simulink model "RBFNN_1221"  (R2018a)
settings: Solver=FixedStepAuto  StartTime=0.0  StopTime=inf  FixedStep=0.001  RelTol=1e-3  EnableMultiTasking=on
undefined symbols (not defined in the file): HIL, j, qc_get_step_size
libraries: dsparch4 x28, quarc_library x17, simulink x7, vrlib x1
(part 1 of 6)
settings Model: SimulationMode=external  ExtModeTrigDuration=10000  Creator=Administrator  LastModifiedBy=ZJUCZ
settings SolverCC: PositivePriorityOrder=on
settings RTWCC: SystemTargetFile=quarc_win64.tlc  TemplateMakefile=quarc_default_tmf  Description=QUARC Win64 Target
settings STFCustomTargetCC: TargetPreCompLibLocation=C:\PROGRA~3\QUARC\lib\2018a\win64\release  TargetLangStandard=C99 (ISO)  ConcurrentExecutionCompliant=on  SystemTargetFile=quarc_win64.tlc
settings GRTTargetCC: TargetPreCompLibLocation=C:\PROGRA~3\QUARC\lib\2018a\win64\release  ParMdlRefBuildCompliant=off  CompOptLevelCompliant=off  CombineOutputUpdateFcns=off  MatFileLogging=off  CPPClassGenCompliant=off  GRTInterface=on  UseToolchainInfoCompliant=off  ExtMode=on  ExtModeMexFile=quarc_comm

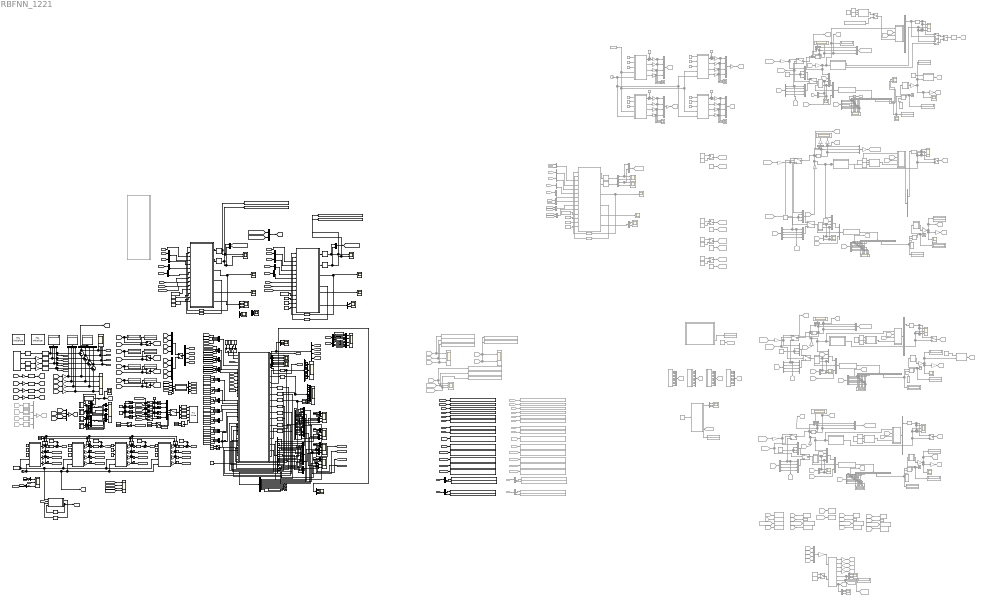
== system RBFNN_1221 ==
  note: 手腕关节的NN控制器
  note: 数据保存区域
  note: 数据传输区
  note: 人工操作区
  note: 轨迹输入区
  note: 向上打是停止运动
  note: 关
      | 节
      | 一
  note: 1关节置零
  note: 关
      | 节
      | 三
  note: 关
      | 节
      | 二
  note: 2关节置零
  note: 3关节置零
  note: 关
      | 节
      | 四
  note: 4关节置零
  note: 左下
  note: 右上
  note: qd
      | e
      | 蓝 FLd QLd
      | 红 FLds1 QLds1
      | 黄 FLda1 QLda1
      | 紫 FLda2 QLda2
      | 绿 QLda3
  note: 主控程序区
  note: 小臂关节的NN控制器
   {,5..7} (4 alike) : Gain  Gain=1/360*2*pi
    {,1..3} (4 alike) : Gain  Commented=on  Gain=1/360*2*pi
     {,1..3} (4 alike) : Gain  Commented=on  Gain=1/360*2*pi
     {4..7} (4 alike) : Gain  Gain=1/360*2*pi
  "  4" : Gain  Commented=on  Gain=-1
  "  5" : Gain  Commented=on
    {6..9} (4 alike) : Gain  Gain=1/360*2*pi
   {1..4} (4 alike) : Gain  Commented=on  Gain=1/360*2*pi
  -25 : Constant  Commented=on  Value=-25
  {1..4} (4 alike) : Gain  Gain=1/360*2*pi
  17.73 : Constant  Commented=on  Value=17.73
  24.22 : Constant  Commented=on  Value=50
  89.3 : Constant  Commented=on  Value=89.3
  Add{,5..7} (4 alike) : Sum  Inputs=++|
  Add{1..4} (4 alike) : Sum  Inputs=+-|
  Analog Filter Design{3..5,7} (4 alike) : dsparch4/Analog Filter Design  Commented=on  method=Butterworth  filttype=Lowpass  N=2  Wlo=30  Whi=80  Rp=2  Rs=40
  Angle from IMU : Subsystem
  Bias : Bias  Bias=-52
  Bias1 : Bias  Bias=+19
  Bias10 : Bias  Bias=-0.5
  Bias11 : Bias  Bias=0.18
  Bias12 : Bias  Bias=0.365
  Bias13 : Bias  Bias=0.21
  Bias14 : Bias  Bias=0.18
  Bias2 : Bias  Bias=-19
  Bias3 : Bias  Bias=-42.6+18+5+2+1-22
  Bias4 : Bias  Bias=-3.5+58
  Bias5 : Bias  Bias=-0.8-1-2
  Bias6 : Bias
  Bias7 : Bias
  Bias8 : Bias  Bias=+0.66
  Bias9 : Bias  Bias=-1.7
  Break : ManualSwitch
  Bus Creator{,1..3} (4 alike) : BusCreator  Commented=on  Inputs=2
  CloseLoop : ManualSwitch  CurrentSetting=0
  Constant{,4..7,11,14,18,31,37,39,44} (12 alike) : Constant  Commented=on  Value=0
  Constant1 : Constant  Commented=on  Value=800
  Constant{2,10,35,41} (4 alike) : Constant  Commented=on  Value=10^3.5
  Constant{12,25,28,60,64,72..73,79..80} (9 alike) : Constant  Value=0
  Constant{3,13,17,36,42} (5 alike) : Constant  Commented=on
  Constant15 : Constant  Value=200-60
  Constant16 : Constant  Commented=on  Value=800
  Constant{9,19,34,40} (4 alike) : Constant  Commented=on  Value=2.5
  Constant20 : Constant  Value=100-50
  Constant21 : Constant  Value=200-50-10
  Constant22 : Constant  Value=100-50
  Constant23 : Constant  Commented=on  Value=-800
  Constant24 : Constant  Value=-0.8
  Constant26 : Constant  Value=-25
  Constant27 : Constant  Value=10
  Constant29 : Constant  Value=5*0
  Constant30 : Constant  Value=0.8
  Constant32 : Constant  Value=100+50
  Constant33 : Constant  Commented=on  Value=800
  Constant38 : Constant  Value=[0;0;0;0]
  Constant43 : Constant  Value=100
  Constant{8,45..46,49,52..53,63,71,78,86} (10 alike) : Constant
  Constant47 : Constant  Value=1e5*5e-3
  Constant48 : Constant  Value=1e5*1e-2
  Constant50 : Constant  Value=1e4
  Constant51 : Constant  Value=1e7
  Constant54 : Constant  Value=100
  Constant55 : Constant  Value=30
  Constant56 : Constant  Value=5e-8
  Constant57 : Constant  Value=6e-8
  Constant58 : Constant  Value=50e-8
  Constant59 : Constant  Value=20e-8
  Constant61 : Constant  Value=240
  Constant62 : Constant  Value=200
  Constant65 : Constant  Value=80
  Constant66 : Constant  Value=80
  Constant67 : Constant  Value=80
  Constant68 : Constant  Value=120
  Constant69 : Constant  Value=100+80+20
  Constant70 : Constant  Value=80-20
  Constant74 : Constant  Commented=on  Value=[5e-7, 8e-4]
  Constant75 : Constant  Commented=on  Value=[ 1, 0.5]
  Constant76 : Constant  Value=3e-3
  Constant77 : Constant  Value=0.5
  Constant81 : Constant  Value=500
  Constant82 : Constant  Commented=on  Value=[1, 1]
  Constant83 : Constant  Commented=on  Value=[500,500]
  Constant84 : Constant  Value=5e-3
  Constant85 : Constant  Value=0.5
  Constant87 : Constant  Value=500
  DIARC_new : MATLAB Function  TreatAsAtomicUnit=on
  Delay : Delay  Commented=on  DelayLength=1
  Delay1 : Delay  DelayLength=1  InitialCondition=[40;60;60;60;25;30;25;20;0;0;0;-10].*2
  Delay10 : Delay  DelayLength=1  InitialCondition=ones(5,1)*0
  Delay11 : Delay  DelayLength=1  InitialCondition=[0,0,0,0,0,0,0,0,0,0,0,0,0,0,0,0,0,0,0,0,0,0,0,0,0,0,0,0,0,0,0,0,0,0,0,0,0]'
  Delay12 : Delay  DelayLength=1  InitialCondition=zeros(5,1)
  Delay13 : Delay  DelayLength=1  InitialCondition=[1e-5,0,0,0,0,0,0,0,0; 0,1e-5,0,0,0,0,0,0,0; 0,0,1e-5,0,0,0,0,0,0; 0,0,0,1e-5,0,0,0,0,0; 0,0,0,0,1e-5,0,0,0,0; 0,0,0,0,0,1e-5,0,0,0; 0,0,0,0,0,0,1e-5,0,0; 0,0,0,0,0,0,0,1e-5,0; 0,0,0,0,0,0,0,0,5e-8]
  Delay{4..5,14..15} (4 alike) : Delay  DelayLength=1  InitialCondition=[0;0;0;0]
  Delay16 : Delay  Commented=on  DelayLength=1  InitialCondition=zeros(5,2)*10-4
  Delay17 : Delay  Commented=on  DelayLength=1  InitialCondition=zeros(5,2)
  Delay18 : Delay  Commented=on  DelayLength=1  InitialCondition=[0,0]
  Delay{3,19,23..24} (4 alike) : Delay  DelayLength=1
  Delay2 : Delay  DelayLength=1  InitialCondition=[0;0;0;0; 0;0;0;0; 2e-10]
  Delay20 : Delay  Commented=on  DelayLength=1  InitialCondition=[0,0]
  Delay21 : Delay  DelayLength=1  InitialCondition=ones(5,1)*1e-4
  Delay22 : Delay  DelayLength=1  InitialCondition=zeros(5,1)
  Delay{6..9} (4 alike) : Delay  DelayLength=1  InitialCondition=[1e-2,0,0; 0,1e-2,0; 0,0,1e-2]
  Demux{,1,3,7} (4 alike) : Demux  Commented=on  Outputs=29
  Demux{2,6,10,18..19,25..28,34,47..48} (12 alike) : Demux
  Demux{11..13,17,49..50} (6 alike) : Demux  Commented=on
  Demux14 : Demux  Commented=on  Outputs=3
  Demux15 : Demux  Commented=on  Outputs=3
  Demux16 : Demux  Commented=on  Outputs=3
  Demux20 : Demux  Outputs=12
  Demux21 : Demux  Outputs=16
  Demux22 : Demux  Outputs=16
  Demux23 : Demux  Outputs=9
  Demux24 : Demux  Outputs=8+4+4
  Demux29 : Demux  Commented=on  Outputs=2
  Demux{30..33,42..45} (8 alike) : Demux  Outputs=[1,1,1,1]
  Demux35 : Demux  Outputs=5
  Demux36 : Demux  Commented=on  Outputs=2
  Demux{37..40} (4 alike) : Demux  Commented=on  Outputs=[1,1,2]
  Demux{4..5,8..9} (4 alike) : Demux  Commented=on  Outputs=27
  Demux41 : Demux  Commented=on  Outputs=2
  Demux46 : Demux  Outputs=2
  Demux51 : Demux  Outputs=5
  Demux52 : Demux  Outputs=5
  Discrete PID Controller1 : simulink/Continuous/PID Controller  Controller=PID  TimeDomain=Continuous-time  SampleTime=-1  IntegratorMethod=Forward Euler  FilterMethod=Backward Euler  Form=Parallel  UseFilter=on  ControllerParametersSource=internal  P=10  I=0  D=0.1  N=2  InitialConditionSource=internal  InitialConditionForIntegrator=0  InitialConditionForFilter=0  ExternalReset=none  IgnoreLimit=on  LimitOutput=off  UpperSaturationLimit=inf  LowerSaturationLimit=-inf  LinearizeAsGain=off  AntiWindupMode=none  Kb=1  TrackingMode=off  Kt=1  PParamMin=[]  PParamMax=[]  IParamMin=[]  IParamMax=[]  DParamMin=[]  DParamMax=[]  NParamMin=[]  NParamMax=[]  KbParamMin=[]  KbParamMax=[]  KtParamMin=[]  KtParamMax=[]  POutMin=[]  POutMax=[]  IOutMin=[]  IOutMax=[]  DOutMin=[]  DOutMax=[]  NOutMin=[]  NOutMax=[]  KbOutMin=[]  KbOutMax=[]  KtOutMin=[]  KtOutMax=[]  IntegratorOutMin=[]  IntegratorOutMax=[]  FilterOutMin=[]  FilterOutMax=[]  SumOutMin=[]  SumOutMax=[]  SumI1OutMin=[]  SumI1OutMax=[]  SumI2OutMin=[]  SumI2OutMax=[]  SumI3OutMin=[]  SumI3OutMax=[]  SumDOutMin=[]  SumDOutMax=[]  SaturationOutMin=[]  SaturationOutMax=[]  IntegratorContinuousStateAttributes=''  IntegratorStateMustResolveToSignalObject=off  IntegratorRTWStateStorageClass=Auto  FilterContinuousStateAttributes=''  FilterStateMustResolveToSignalObject=off  FilterRTWStateStorageClass=Auto  DifferentiatorICPrevScaledInput=0  DifferentiatorOutMin=[]  DifferentiatorOutMax=[]  FilterDiffOutCoefMin=[]  FilterDiffOutCoefMax=[]  SumDenOutMin=[]  SumDenOutMax=[]  SumNumOutMin=[]  SumNumOutMax=[]  ReciprocalOutMin=[]  ReciprocalOutMax=[]  DivideOutMin=[]  DivideOutMax=[]  TunerSelectOption=Transfer Function Based (PID Tuner App)
  Discrete PID Controller2 : simulink/Continuous/PID Controller  Controller=PID  TimeDomain=Continuous-time  SampleTime=-1  IntegratorMethod=Forward Euler  FilterMethod=Backward Euler  Form=Parallel  UseFilter=on  ControllerParametersSource=internal  P=8  I=0  D=0.001  N=1e2  InitialConditionSource=internal  InitialConditionForIntegrator=0  InitialConditionForFilter=0  ExternalReset=none  IgnoreLimit=on  LimitOutput=off  UpperSaturationLimit=inf  LowerSaturationLimit=-inf  LinearizeAsGain=off  AntiWindupMode=none  Kb=1  TrackingMode=off  Kt=1  PParamMin=[]  PParamMax=[]  IParamMin=[]  IParamMax=[]  DParamMin=[]  DParamMax=[]  NParamMin=[]  NParamMax=[]  KbParamMin=[]  KbParamMax=[]  KtParamMin=[]  KtParamMax=[]  POutMin=[]  POutMax=[]  IOutMin=[]  IOutMax=[]  DOutMin=[]  DOutMax=[]  NOutMin=[]  NOutMax=[]  KbOutMin=[]  KbOutMax=[]  KtOutMin=[]  KtOutMax=[]  IntegratorOutMin=[]  IntegratorOutMax=[]  FilterOutMin=[]  FilterOutMax=[]  SumOutMin=[]  SumOutMax=[]  SumI1OutMin=[]  SumI1OutMax=[]  SumI2OutMin=[]  SumI2OutMax=[]  SumI3OutMin=[]  SumI3OutMax=[]  SumDOutMin=[]  SumDOutMax=[]  SaturationOutMin=[]  SaturationOutMax=[]  IntegratorContinuousStateAttributes=''  IntegratorStateMustResolveToSignalObject=off  IntegratorRTWStateStorageClass=Auto  FilterContinuousStateAttributes=''  FilterStateMustResolveToSignalObject=off  FilterRTWStateStorageClass=Auto  DifferentiatorICPrevScaledInput=0  DifferentiatorOutMin=[]  DifferentiatorOutMax=[]  FilterDiffOutCoefMin=[]  FilterDiffOutCoefMax=[]  SumDenOutMin=[]  SumDenOutMax=[]  SumNumOutMin=[]  SumNumOutMax=[]  ReciprocalOutMin=[]  ReciprocalOutMax=[]  DivideOutMin=[]  DivideOutMax=[]  TunerSelectOption=Transfer Function Based (PID Tuner App)
  Discrete PID Controller3 : simulink/Continuous/PID Controller  Controller=PID  TimeDomain=Continuous-time  SampleTime=-1  IntegratorMethod=Forward Euler  FilterMethod=Backward Euler  Form=Parallel  UseFilter=on  ControllerParametersSource=internal  P=15  I=0  D=0.003  N=2  InitialConditionSource=internal  InitialConditionForIntegrator=0  InitialConditionForFilter=0  ExternalReset=none  IgnoreLimit=on  LimitOutput=off  UpperSaturationLimit=inf  LowerSaturationLimit=-inf  LinearizeAsGain=off  AntiWindupMode=none  Kb=1  TrackingMode=off  Kt=1  PParamMin=[]  PParamMax=[]  IParamMin=[]  IParamMax=[]  DParamMin=[]  DParamMax=[]  NParamMin=[]  NParamMax=[]  KbParamMin=[]  KbParamMax=[]  KtParamMin=[]  KtParamMax=[]  POutMin=[]  POutMax=[]  IOutMin=[]  IOutMax=[]  DOutMin=[]  DOutMax=[]  NOutMin=[]  NOutMax=[]  KbOutMin=[]  KbOutMax=[]  KtOutMin=[]  KtOutMax=[]  IntegratorOutMin=[]  IntegratorOutMax=[]  FilterOutMin=[]  FilterOutMax=[]  SumOutMin=[]  SumOutMax=[]  SumI1OutMin=[]  SumI1OutMax=[]  SumI2OutMin=[]  SumI2OutMax=[]  SumI3OutMin=[]  SumI3OutMax=[]  SumDOutMin=[]  SumDOutMax=[]  SaturationOutMin=[]  SaturationOutMax=[]  IntegratorContinuousStateAttributes=''  IntegratorStateMustResolveToSignalObject=off  IntegratorRTWStateStorageClass=Auto  FilterContinuousStateAttributes=''  FilterStateMustResolveToSignalObject=off  FilterRTWStateStorageClass=Auto  DifferentiatorICPrevScaledInput=0  DifferentiatorOutMin=[]  DifferentiatorOutMax=[]  FilterDiffOutCoefMin=[]  FilterDiffOutCoefMax=[]  SumDenOutMin=[]  SumDenOutMax=[]  SumNumOutMin=[]  SumNumOutMax=[]  ReciprocalOutMin=[]  ReciprocalOutMax=[]  DivideOutMin=[]  DivideOutMax=[]  TunerSelectOption=Transfer Function Based (PID Tuner App)
  Discrete PID Controller5 : simulink/Continuous/PID Controller  Controller=PID  TimeDomain=Continuous-time  SampleTime=-1  IntegratorMethod=Forward Euler  FilterMethod=Backward Euler  Form=Parallel  UseFilter=on  ControllerParametersSource=internal  P=5.5  I=0  D=0.003  N=100  InitialConditionSource=internal  InitialConditionForIntegrator=0  InitialConditionForFilter=0  ExternalReset=none  IgnoreLimit=on  LimitOutput=off  UpperSaturationLimit=inf  LowerSaturationLimit=-inf  LinearizeAsGain=off  AntiWindupMode=none  Kb=1  TrackingMode=off  Kt=1  PParamMin=[]  PParamMax=[]  IParamMin=[]  IParamMax=[]  DParamMin=[]  DParamMax=[]  NParamMin=[]  NParamMax=[]  KbParamMin=[]  KbParamMax=[]  KtParamMin=[]  KtParamMax=[]  POutMin=[]  POutMax=[]  IOutMin=[]  IOutMax=[]  DOutMin=[]  DOutMax=[]  NOutMin=[]  NOutMax=[]  KbOutMin=[]  KbOutMax=[]  KtOutMin=[]  KtOutMax=[]  IntegratorOutMin=[]  IntegratorOutMax=[]  FilterOutMin=[]  FilterOutMax=[]  SumOutMin=[]  SumOutMax=[]  SumI1OutMin=[]  SumI1OutMax=[]  SumI2OutMin=[]  SumI2OutMax=[]  SumI3OutMin=[]  SumI3OutMax=[]  SumDOutMin=[]  SumDOutMax=[]  SaturationOutMin=[]  SaturationOutMax=[]  IntegratorContinuousStateAttributes=''  IntegratorStateMustResolveToSignalObject=off  IntegratorRTWStateStorageClass=Auto  FilterContinuousStateAttributes=''  FilterStateMustResolveToSignalObject=off  FilterRTWStateStorageClass=Auto  DifferentiatorICPrevScaledInput=0  DifferentiatorOutMin=[]  DifferentiatorOutMax=[]  FilterDiffOutCoefMin=[]  FilterDiffOutCoefMax=[]  SumDenOutMin=[]  SumDenOutMax=[]  SumNumOutMin=[]  SumNumOutMax=[]  ReciprocalOutMin=[]  ReciprocalOutMax=[]  DivideOutMin=[]  DivideOutMax=[]  TunerSelectOption=Transfer Function Based (PID Tuner App)
  Display{1,8,23,25..27,32..33} (8 alike) : Display
  Display{3,5..6,12..14,16..19,21,24,28..29,31,34} (16 alike) : Display  Commented=on
  Divide{,1..3} (4 alike) : Product  Commented=on  Inputs=*/
  From : From  Commented=on  GotoTag=q1
  From1 : From  Commented=on  GotoTag=QL_1
  From107 : From  Commented=on  GotoTag=q1
  From108 : From  Commented=on  GotoTag=q2
  From109 : From  Commented=on  GotoTag=q3
  From11 : From  Commented=on  GotoTag=dx_3
  From110 : From  Commented=on  GotoTag=q4
  From14 : From  Commented=on  GotoTag=Theta1
  From140 : From  Commented=on  GotoTag=P_i
  From141 : From  Commented=on  GotoTag=P_o
  From142 : From  Commented=on  GotoTag=z2
  From143 : From  Commented=on  GotoTag=z3
  From144 : From  Commented=on  GotoTag=z1
  From149 : From  Commented=on  GotoTag=qd4_dot
  From153 : From  Commented=on  GotoTag=qd4_ddot
  From154 : From  Commented=on  GotoTag=qd4
  From166 : From  Commented=on  GotoTag=z2
  From167 : From  Commented=on  GotoTag=e3
  From168 : From  Commented=on  GotoTag=z3
  From169 : From  Commented=on  GotoTag=P_i
  From17 : From  Commented=on  GotoTag=P1
  From170 : From  Commented=on  GotoTag=P_o
  From171 : From  Commented=on  GotoTag=qd4_dot
  From172 : From  Commented=on  GotoTag=qd3_dddot
  From173 : From  Commented=on  GotoTag=qd3
  From174 : From  Commented=on  GotoTag=e4
  From175 : From  Commented=on  GotoTag=qd4
  From176 : From  Commented=on  GotoTag=qd3_dot
  From177 : From  Commented=on  GotoTag=qd4_dddot
  From19 : From  Commented=on  GotoTag=xv_1
  From199 : From  Commented=on  GotoTag=e3
  From2 : From  Commented=on  GotoTag=q3
  From20 : From  Commented=on  GotoTag=Theta2
  From200 : From  Commented=on  GotoTag=e4
  From201 : From  Commented=on  GotoTag=arc3
  From202 : From  Commented=on  GotoTag=arc4
  From203 : From  Commented=on  GotoTag=joint3_Fld
  From204 : From  Commented=on  GotoTag=joint4_Fld
  From205 : From  Commented=on  GotoTag=joint3_Qld
  From206 : From  Commented=on  GotoTag=joint4_Qld
  From207 : From  Commented=on  GotoTag=q3
  From208 : From  Commented=on  GotoTag=q4
  From209 : From  Commented=on  GotoTag=qd3
  From21 : From  Commented=on  GotoTag=P2
  From210 : From  Commented=on  GotoTag=qd4
  From211 : From  Commented=on  GotoTag=P_i
  From212 : From  Commented=on  GotoTag=P_o
  From213 : From  Commented=on  GotoTag=qd3_dot
  From214 : From  Commented=on  GotoTag=qd4_dot
  From22 : From  Commented=on  GotoTag=tracking_result_2
  From23 : From  Commented=on  GotoTag=xv_2
  From27 : From  Commented=on  GotoTag=dx_1
  From29 : From  Commented=on  GotoTag=QL_3
  From3 : From  Commented=on  GotoTag=Theta1
  From31 : From  Commented=on  GotoTag=Theta3
  From32 : From  Commented=on  GotoTag=Theta3
  From33 : From  Commented=on  GotoTag=P3
  From34 : From  Commented=on  GotoTag=tracking_result_3
  From35 : From  Commented=on  GotoTag=xv_3
  From36 : From  Commented=on  GotoTag=dx_2
  From37 : From  Commented=on  GotoTag=q2
  From38 : From  Commented=on  GotoTag=QL_2
  From40 : From  Commented=on  GotoTag=Theta2
  From50 : From  Commented=on  GotoTag=setzero1
  From51 : From  Commented=on  GotoTag=setzero2
  From52 : From  Commented=on  GotoTag=setzero3
  From57 : From  Commented=on  GotoTag=setvalue1
  From58 : From  Commented=on  GotoTag=setvalue2
  From59 : From  Commented=on  GotoTag=setvalue3
  From60 : From  Commented=on  GotoTag=para1
  From61 : From  Commented=on  GotoTag=para2
  From62 : From  Commented=on  GotoTag=para3
  From63 : From  Commented=on  GotoTag=dx_4
  From64 : From  Commented=on  GotoTag=q4
  From65 : From  Commented=on  GotoTag=QL_4
  From66 : From  Commented=on  GotoTag=Theta4
  From67 : From  Commented=on  GotoTag=setzero4
  From68 : From  Commented=on  GotoTag=setvalue4
  From69 : From  Commented=on  GotoTag=para4
  From74 : From  Commented=on  GotoTag=Theta4
  From75 : From  Commented=on  GotoTag=P4
  From76 : From  Commented=on  GotoTag=tracking_result_4
  From77 : From  Commented=on  GotoTag=xv_4
  From8 : From  Commented=on  GotoTag=tracking_result_1
  From82 : From  Commented=on  GotoTag=errorxyz
  From83 : From  Commented=on  GotoTag=J1_new
  From84 : From  Commented=on  GotoTag=J2_new
  From85 : From  Commented=on  GotoTag=J3_new
  From86 : From  Commented=on  GotoTag=XYZ
  From87 : From  Commented=on  GotoTag=qr4
  From88 : From  Commented=on  GotoTag=qr2
  From89 : From  Commented=on  GotoTag=qr3
  From90 : From  Commented=on  GotoTag=qr1
  From91 : From  Commented=on  GotoTag=J4_new
  Gain{,6..7,16,23,33..36} (9 alike) : Gain  Gain=180/pi
  Gain{1,4,13,20} (4 alike) : Gain  Commented=on
  Gain{3,8..11,15,22,24..28} (12 alike) : Gain  Commented=on  Gain=pi/180
  Gain{12,30..32} (4 alike) : Gain  Gain=-1
  Gain{2,5,14,21} (4 alike) : Gain  Commented=on  Gain=10
  Gain17 : Gain  Commented=on  Gain=-1
  Gain18 : Gain  Commented=on  Gain=-1
  Gain19 : Gain  Commented=on  Gain=-1
  Gain29 : Gain  Commented=on  Gain=180/pi
  Goto : Goto  Commented=on  GotoTag=J1
  Goto10 : Goto  Commented=on  GotoTag=Theta3
  Goto106 : Goto  Commented=on  GotoTag=q_dot
  Goto120 : Goto  Commented=on  GotoTag=RBFNN
  Goto15 : Goto  Commented=on  GotoTag=QL_1
  Goto16 : Goto  Commented=on  GotoTag=dx_1
  Goto17 : Goto  Commented=on  GotoTag=tracking_result_1
  Goto18 : Goto  Commented=on  GotoTag=xv_1
  Goto19 : Goto  Commented=on  GotoTag=tracking_result_3
  Goto20 : Goto  Commented=on  GotoTag=xv_3
  Goto21 : Goto  Commented=on  GotoTag=Theta2
  Goto23 : Goto  Commented=on  GotoTag=QL_3
  Goto24 : Goto  Commented=on  GotoTag=J1_new
  Goto26 : Goto  Commented=on  GotoTag=dx_3
  Goto28 : Goto  Commented=on  GotoTag=tracking_result_2
  Goto29 : Goto  Commented=on  GotoTag=xv_2
  Goto3 : Goto  Commented=on  GotoTag=P1
  Goto30 : Goto  Commented=on  GotoTag=QL_2
  Goto31 : Goto  Commented=on  GotoTag=dx_2
  Goto32 : Goto  Commented=on  GotoTag=P2
  Goto33 : Goto  Commented=on  GotoTag=arc1
  Goto34 : Goto  Commented=on  GotoTag=arc2
  Goto35 : Goto  Commented=on  GotoTag=arc3
  Goto40 : Goto  Commented=on  GotoTag=setzero1
  Goto41 : Goto  Commented=on  GotoTag=setzero2
  Goto42 : Goto  Commented=on  GotoTag=setzero3
  Goto43 : Goto  Commented=on  GotoTag=xd1
  Goto44 : Goto  Commented=on  GotoTag=xd3
  Goto45 : Goto  Commented=on  GotoTag=xd2
  Goto47 : Goto  Commented=on  GotoTag=setvalue1
  Goto48 : Goto  Commented=on  GotoTag=setvalue2
  Goto49 : Goto  Commented=on  GotoTag=setvalue3
  Goto5 : Goto  Commented=on  GotoTag=error
  Goto50 : Goto  Commented=on  GotoTag=para1
  Goto51 : Goto  Commented=on  GotoTag=para2
  Goto52 : Goto  Commented=on  GotoTag=para3
  Goto53 : Goto  Commented=on  GotoTag=Theta4
  Goto54 : Goto  Commented=on  GotoTag=tracking_result_4
  Goto55 : Goto  Commented=on  GotoTag=xv_4
  Goto56 : Goto  Commented=on  GotoTag=QL_4
  Goto57 : Goto  Commented=on  GotoTag=dx_4
  Goto58 : Goto  Commented=on  GotoTag=P4
  Goto59 : Goto  Commented=on  GotoTag=arc4
  Goto60 : Goto  Commented=on  GotoTag=xd4
  Goto62 : Goto  Commented=on  GotoTag=setzero4
  Goto63 : Goto  Commented=on  GotoTag=setvalue4
  Goto67 : Goto  Commented=on  GotoTag=para4
  Goto68 : Goto  Commented=on  GotoTag=J2
  Goto69 : Goto  Commented=on  GotoTag=J3
  Goto7 : Goto  Commented=on  GotoTag=Theta1
  Goto70 : Goto  Commented=on  GotoTag=J4
  Goto71 : Goto  Commented=on  GotoTag=error
  Goto72 : Goto  Commented=on  GotoTag=error
  Goto73 : Goto  Commented=on  GotoTag=XYZ
  Goto74 : Goto  Commented=on  GotoTag=qr1
  Goto75 : Goto  Commented=on  GotoTag=qr2
  Goto76 : Goto  Commented=on  GotoTag=qr3
  Goto77 : Goto  Commented=on  GotoTag=qr4
  Goto78 : Goto  Commented=on  GotoTag=errorxyz
  Goto79 : Goto  Commented=on  GotoTag=e2
  Goto8 : Goto  Commented=on  GotoTag=P3
  Goto80 : Goto  Commented=on  GotoTag=e1
  Goto81 : Goto  Commented=on  GotoTag=e3
  Goto82 : Goto  Commented=on  GotoTag=e4
  Goto83 : Goto  Commented=on  GotoTag=J2_new
  Goto87 : Goto  Commented=on  GotoTag=J3_new
  Goto88 : Goto  Commented=on  GotoTag=J4_new
  HIL Initialize : quarc_library/Data Acquisition/Generic/Configuration/HIL Initialize  object_name=HIL-1  board_type=qpid_e  board_number=0  board_options=enc0_dir=0;enc0_filter=1;enc0_a=1;enc0_b=1;enc0_z=0;enc0_reload=0;enc1_dir=0;enc1_filter=1;enc1_a=1;enc1_b=1;enc1_z=0;enc1_reload=0;enc2_dir=0;enc2_filter=1;enc2_a=1;enc2_b=1;enc2_z=0;enc2_reload=0;enc3_dir=0;enc3_filter=1;enc3_a=1;enc3_b=1;enc3_z=0;enc3_reload=0;enc4_dir=0;enc4_filter=1;enc4_a=1;enc4_b=1;enc4_z=0;enc4_reload=0;enc5_dir=0;enc5_filter=1;enc5_a=1;enc5_b=1;enc5_z=0;enc5_reload=0;enc6_dir=0;enc6_filter=1;enc6_a=1;enc6_b=1;enc6_z=0;enc6_reload=0;enc7_dir=0;enc7_filter=1;enc7_a=1;enc7_b=1;enc7_z=0;enc7_reload=0;ext_int_polarity=0;fuse_polarity=0;convert_polarity=0;watchdog_polarity=0;ext_int_watchdog=0;fuse_watchdog=0;trig1_watchdog=0;watchdog_to_trig1=0;watchdog_to_trig2=0;counter_to_trig0=0;trigger_adcs=0;latch_on_adc=0;pwm_immediate=0  exclusive=off  active=on  hardware_clocks=[0:16]  clock_modes=[]  initial_clock_frequencies=[]  set_clock_params_at_start=off  set_clock_params_at_switch_in=off  set_clock_frequencies_at_start=off  set_clock_frequencies_at_switch_in=off  analog_input_channels=[0:7]  analog_input_configurations=[]  analog_input_maximums=10  analog_input_minimums=-10  set_analog_input_params_at_start=off  set_analog_input_params_at_switch_in=off  analog_output_channels=[0:7]  analog_output_maximums=10  analog_output_minimums=-10  initial_analog_outputs=[0]  final_analog_outputs=[0]  watchdog_analog_outputs=0  set_analog_output_params_at_start=off  set_analog_output_params_at_switch_in=off  set_analog_outputs_at_start=on  set_analog_outputs_at_switch_in=off  set_analog_outputs_at_terminate=on  set_analog_outputs_at_switch_out=off  set_analog_outputs_on_watchdog=off  digital_input_channels=[]  digital_output_channels=[]  digital_output_configuration=[]  initial_digital_outputs=[1]  final_digital_outputs=[1]  watchdog_digital_outputs=[2]  set_digital_output_params_at_start=off  set_digital_output_params_at_switch_in=off  set_digital_outputs_at_start=on  set_digital_outputs_at_switch_in=off  set_digital_outputs_at_terminate=on  set_digital_outputs_at_switch_out=off  set_digital_outputs_on_watchdog=off  encoder_channels=[0:7]  quadrature=[4]  encoder_filter_frequency=40e6/1  initial_encoder_counts=[0]  set_encoder_params_at_start=on  set_encoder_params_at_switch_in=off  set_encoder_counts_at_start=on  set_encoder_counts_at_switch_in=off  pwm_channels=[0:7]  pwm_modes=0  pwm_frequency=40e6/4096  pwm_configuration=[0]  pwm_alignment=[0]  pwm_polarity=[1]  pwm_leading_deadband=[0]  pwm_trailing_deadband=[0]  initial_pwm_outputs=[0]  final_pwm_outputs=[0]  watchdog_pwm_outputs=[0]  set_pwm_params_at_start=on  set_pwm_params_at_switch_in=off  set_pwm_outputs_at_start=on  set_pwm_outputs_at_switch_in=off  set_pwm_outputs_at_terminate=on  set_pwm_outputs_at_switch_out=off  set_pwm_outputs_on_watchdog=off  other_output_channels=[]  initial_other_outputs=[]  final_other_outputs=[]  watchdog_other_outputs=[]  set_other_outputs_at_start=off  set_other_outputs_at_switch_in=off  set_other_outputs_at_terminate=off  set_other_outputs_at_switch_out=off  set_other_outputs_on_watchdog=off
  HIL Initialize2 : quarc_library/Data Acquisition/Generic/Configuration/HIL Initialize  object_name=HIL-2  board_type=q8_usb  board_number=0  board_options=update_rate=fast;ext_int_polarity=0;convert_polarity=1;watchdog_polarity=0;ext_int_watchdog=0;use_convert=0;pwm_immediate=0;decimation=1  exclusive=off  active=on  hardware_clocks=[0:2]  clock_modes=[]  initial_clock_frequencies=[]  set_clock_params_at_start=off  set_clock_params_at_switch_in=off  set_clock_frequencies_at_start=off  set_clock_frequencies_at_switch_in=off  analog_input_channels=[0:7]  analog_input_configurations=[]  analog_input_maximums=10  analog_input_minimums=-10  set_analog_input_params_at_start=on  set_analog_input_params_at_switch_in=off  analog_output_channels=[0:7]  analog_output_maximums=10  analog_output_minimums=-10  initial_analog_outputs=[0]  final_analog_outputs=[0]  watchdog_analog_outputs=0  set_analog_output_params_at_start=on  set_analog_output_params_at_switch_in=off  set_analog_outputs_at_start=on  set_analog_outputs_at_switch_in=off  set_analog_outputs_at_terminate=on  set_analog_outputs_at_switch_out=off  set_analog_outputs_on_watchdog=off  digital_input_channels=[]  digital_output_channels=[]  digital_output_configuration=[]  initial_digital_outputs=[1]  final_digital_outputs=[1]  watchdog_digital_outputs=[1]  set_digital_output_params_at_start=off  set_digital_output_params_at_switch_in=off  set_digital_outputs_at_start=on  set_digital_outputs_at_switch_in=off  set_digital_outputs_at_terminate=on  set_digital_outputs_at_switch_out=off  set_digital_outputs_on_watchdog=off  encoder_channels=[0:7]  quadrature=[4]  encoder_filter_frequency=[]  initial_encoder_counts=[0]  set_encoder_params_at_start=on  set_encoder_params_at_switch_in=off  set_encoder_counts_at_start=on  set_encoder_counts_at_switch_in=off  pwm_channels=[0:7]  pwm_modes=0  pwm_frequency=99.532799999999995e6/4095  pwm_configuration=[0]  pwm_alignment=[0]  pwm_polarity=[1]  pwm_leading_deadband=[0]  pwm_trailing_deadband=[0]  initial_pwm_outputs=[0]  final_pwm_outputs=[0]  watchdog_pwm_outputs=[0]  set_pwm_params_at_start=on  set_pwm_params_at_switch_in=off  set_pwm_outputs_at_start=on  set_pwm_outputs_at_switch_in=off  set_pwm_outputs_at_terminate=on  set_pwm_outputs_at_switch_out=off  set_pwm_outputs_on_watchdog=off  other_output_channels=[]  initial_other_outputs=[]  final_other_outputs=[]  watchdog_other_outputs=[]  set_other_outputs_at_start=off  set_other_outputs_at_switch_in=off  set_other_outputs_at_terminate=off  set_other_outputs_at_switch_out=off  set_other_outputs_on_watchdog=off
  HIL Read Analog : quarc_library/Data Acquisition/Generic/Immediate I//O/HIL Read Analog  object_name=HIL-1  channels=[0]  sample_time=qc_get_step_size  active=on  vector_output=off
  HIL Write : quarc_library/Data Acquisition/Generic/Immediate I//O/HIL Write  object_name=HIL-1  analog_channels=[1:5]  pwm_channels=[]  digital_channels=[]  other_channels=[]  sample_time=-1  active=off  vector_input=off
  J1_P2P(the out is degree°) : MATLAB Function  TreatAsAtomicUnit=on
  J2_P2P(the out is degree°) : MATLAB Function  TreatAsAtomicUnit=on
  J3_P2P(the out is degree°) : MATLAB Function  TreatAsAtomicUnit=on
  J4_P2P(the out is degree°) : MATLAB Function  TreatAsAtomicUnit=on
  K_1 : Mux
  K_2 : Mux
  K_3 : Mux
  Look_J{1..4} (4 alike) : Scope  NumInputPorts=4
  Look_q qdot : Scope  NumInputPorts=4
  Look_q1dot : Scope  NumInputPorts=3
  MATLAB Function : MATLAB Function  Commented=on  TreatAsAtomicUnit=on
  MATLAB Function1 : MATLAB Function  Commented=on  TreatAsAtomicUnit=on
  MATLAB Function10 : MATLAB Function  Commented=on  TreatAsAtomicUnit=on
  MATLAB Function7 : MATLAB Function  Commented=on  TreatAsAtomicUnit=on
  MATLAB Function8 : MATLAB Function  Commented=on  TreatAsAtomicUnit=on
  MATLAB Function9 : MATLAB Function  Commented=on  TreatAsAtomicUnit=on
  MPa2Pa : Gain  Gain=1e6
  MPa2Pa1 : Gain  Gain=1e6
  MPa2Pa2 : Gain  Gain=1e6
  Manual Switch{,1..2,6..7,10,15..16,18} (9 alike) : ManualSwitch  Commented=on
  Manual Switch{5,9,11..13,20} (6 alike) : ManualSwitch  CurrentSetting=0
  Manual Switch14 : ManualSwitch  Commented=on  CurrentSetting=0
  Manual Switch{4,8,17,21..25} (8 alike) : ManualSwitch
  Manual Switch19 : ManualSwitch  Commented=on  CurrentSetting=0
  Manual Switch3 : ManualSwitch  Commented=on  CurrentSetting=0
  Multiply : Product
  Multiply1 : Product
  Mux{,2,7..10,13,18,24..25,34..35,38,59,84} (15 alike) : Mux  Commented=on
  Mux{1,4,11..12,19..21,31} (8 alike) : Mux  Commented=on  Inputs=3
  Mux{6,14,22,32} (4 alike) : Mux  Commented=on  Inputs=7
  Mux{5,15,23,33,86,88..90} (8 alike) : Mux  Commented=on  Inputs=2
  Mux{16..17,26..28,37,39..58,61} (27 alike) : Mux
  Mux{3,29..30,36} (4 alike) : Mux  Commented=on  Inputs=11
  Mux{60,62..72,77..83,85,87} (21 alike) : Mux  Inputs=2
  Mux{73..76} (4 alike) : Mux  Inputs=3
  Nan Switch : Subsystem
  Obs Para Generator1 : MATLAB Function  Commented=on  TreatAsAtomicUnit=on
  Obs Para Generator2 : MATLAB Function  Commented=on  TreatAsAtomicUnit=on
  Obs Para Generator3 : MATLAB Function  Commented=on  TreatAsAtomicUnit=on
  Obs Para Generator4 : MATLAB Function  Commented=on  TreatAsAtomicUnit=on
  P1 : Subsystem
  P2 : Subsystem
  P3 : Subsystem
  P4 : Subsystem
  PID/ARC1 : ManualSwitch  CurrentSetting=0
  PID/ARC2 : ManualSwitch
  PID/ARC3 : ManualSwitch  CurrentSetting=0
  PID/ARC4 : ManualSwitch  CurrentSetting=0
  P_scope1 : Scope  NumInputPorts=4
  P_scope2 : Scope
  Product{,1..15} (16 alike) : Product
  RBFNN_muti : MATLAB Function  Commented=on  TreatAsAtomicUnit=on
  RBFNN_smallarm : MATLAB Function  TreatAsAtomicUnit=on
  RBFNN_wrist : MATLAB Function  TreatAsAtomicUnit=on
  RBFNN_wrist1 : MATLAB Function  Commented=on  TreatAsAtomicUnit=on
  S-Function1 : S-Function  Commented=on  FunctionName=ARC_BACKSTEPPING3  SFunctionDeploymentMode=off  EnableBusSupport=off
  S-Function2 : S-Function  Commented=on  FunctionName=ARC_BACKSTEPPING  SFunctionDeploymentMode=off  EnableBusSupport=off
  S-Function3 : S-Function  Commented=on  FunctionName=ARC_BACKSTEPPING2  SFunctionDeploymentMode=off  EnableBusSupport=off
  S-Function4 : S-Function  Commented=on  FunctionName=ARC_BACKSTEPPING4  SFunctionDeploymentMode=off  EnableBusSupport=off
  Scope{,3..4,12,14,25..27} (8 alike) : Scope  Commented=on  NumInputPorts=2
  Scope{1,13,17,22} (4 alike) : Scope  NumInputPorts=4
  Scope{2,10..11,16,18} (5 alike) : Scope  Commented=on  NumInputPorts=3
  Scope{8..9,15,20,23..24} (6 alike) : Scope  Commented=on
  Scope{7,19,21,28..29} (5 alike) : Scope
  Scope30 : Scope  NumInputPorts=2
  Scope31 : Scope  NumInputPorts=2
  Scope32 : Scope  NumInputPorts=5
  Scope33 : Scope  NumInputPorts=5
  Scope5 : Scope  NumInputPorts=2
  Scope6 : Scope  NumInputPorts=5
  Subsystem : Subsystem  Commented=on
  Subsystem1 : Subsystem  Commented=on
  Subsystem2 : Subsystem  Commented=on
  Subsystem3 : Subsystem  Commented=on
  Subsystem4 : Subsystem  Commented=on
  Subsystem5 : Subsystem  Commented=on
  Subsystem6 : Subsystem  Commented=on
  Subsystem7 : Subsystem  Commented=on
  Subsystem8 : Subsystem  Commented=on
  Subsystem9 : Subsystem  Commented=on
  Sum{1,3,5..6} (4 alike) : Sum  Commented=on  Inputs=+-|
  Switch{,1..4,10,12..13} (8 alike) : Switch  Commented=on  Criteria=u2 ~= 0
  Switch{6..9,11} (5 alike) : Switch
  Switch5 : ManualSwitch  CurrentSetting=0
  To File : ToFile  Commented=on  Filename=tracking_result_1  MatrixName=tracking_result
  To File1 : ToFile  Commented=on  Filename=p_1  MatrixName=p
  To File10 : ToFile  Commented=on  Filename=tracking_result_3  MatrixName=tracking_result
  To File11 : ToFile  Commented=on  Filename=theta_3  MatrixName=theta
  To File12 : ToFile  Commented=on  Filename=xv_3  MatrixName=xv
  To File13 : ToFile  Commented=on  Filename=p_3  MatrixName=p
  To File14 : ToFile  Commented=on  Filename=C:\Users\ZJUCZ\Desktop\RBFNN_EXPERMENT\joint4_e3  MatrixName=joint4_e3
  To File15 : ToFile  Commented=on  Filename=tracking_result_4  MatrixName=tracking_result
  To File16 : ToFile  Commented=on  Filename=theta_4  MatrixName=theta
  To File17 : ToFile  Commented=on  Filename=xv_4  MatrixName=xv
  To File18 : ToFile  Commented=on  Filename=p_4  MatrixName=p
  To File19 : ToFile  Commented=on  Filename=C:\Users\ZJUCZ\Desktop\RBFNN_EXPERMENT\joint4_qd  MatrixName=joint4_qd
  To File2 : ToFile  Commented=on  Filename=theta_1  MatrixName=theta
  To File20 : ToFile  Commented=on  Filename=xyz
  To File21 : ToFile  Commented=on  Filename=errorxyz
  To File22 : ToFile  Commented=on  Filename=C:\Users\ZJUCZ\Desktop\RBFNN_EXPERMENT\joint4_pi  MatrixName=joint4_pi
  To File23 : ToFile  Commented=on  Filename=C:\Users\ZJUCZ\Desktop\RBFNN_EXPERMENT\joint4_po  MatrixName=joint4_po
  To File24 : ToFile  Commented=on  Filename=C:\Users\ZJUCZ\Desktop\RBFNN_EXPERMENT\joint4_qd_dot  MatrixName=joint4_qd_dot
  To File25 : ToFile  Commented=on  Filename=C:\Users\ZJUCZ\Desktop\RBFNN_EXPERMENT\joint4_qd_ddot  MatrixName=joint4_qd_ddot
  To File26 : ToFile  Filename=C:\Users\ZJUCZ\Desktop\RBFNN_EXPERMENT\data\joint_3_nndrc_error.mat  MatrixName=joint_3_nndrc_error
  To File27 : ToFile  Filename=C:\Users\ZJUCZ\Desktop\RBFNN_EXPERMENT\data\joint_4_nndrc_error.mat  MatrixName=joint_4_nndrc_error
  To File28 : ToFile  Filename=C:\Users\ZJUCZ\Desktop\RBFNN_EXPERMENT\data\joint_3_nndrc_qd.mat  MatrixName=joint_3_nndrc_qd
  To File29 : ToFile  Filename=C:\Users\ZJUCZ\Desktop\RBFNN_EXPERMENT\data\joint_4_nndrc_qd.mat  MatrixName=joint_4_nndrc_qd
  To File3 : ToFile  Commented=on  Filename=xv_1  MatrixName=xv
  To File30 : ToFile  Filename=C:\Users\ZJUCZ\Desktop\RBFNN_EXPERMENT\data\joint_4_nndrc_P_i.mat  MatrixName=joint_4_nndrc_P_i
  To File31 : ToFile  Filename=C:\Users\ZJUCZ\Desktop\RBFNN_EXPERMENT\data\joint_3_nndrc_P_i.mat  MatrixName=joint_3_nndrc_P_i
  To File32 : ToFile  Filename=C:\Users\ZJUCZ\Desktop\RBFNN_EXPERMENT\data\joint_4_nndrc_P_o.mat  MatrixName=joint_4_nndrc_P_o
  To File33 : ToFile  Filename=C:\Users\ZJUCZ\Desktop\RBFNN_EXPERMENT\data\joint_3_nndrc_P_o.mat  MatrixName=joint_3_nndrc_P_o
  To File34 : ToFile  Filename=C:\Users\ZJUCZ\Desktop\RBFNN_EXPERMENT\data\joint_3_nndrc_U.mat  MatrixName=joint_3_nndrc_U
  To File35 : ToFile  Filename=C:\Users\ZJUCZ\Desktop\RBFNN_EXPERMENT\data\joint_4_nndrc_U.mat  MatrixName=joint_4_nndrc_U
  To File36 : ToFile  Filename=C:\Users\ZJUCZ\Desktop\RBFNN_EXPERMENT\data\joint_3_nndrc_Fld.mat  MatrixName=joint_3_nndrc_Fld
  To File37 : ToFile  Filename=C:\Users\ZJUCZ\Desktop\RBFNN_EXPERMENT\data\joint_3_nndrc_Qld.mat  MatrixName=joint_3_nndrc_Qld
  To File38 : ToFile  Filename=C:\Users\ZJUCZ\Desktop\RBFNN_EXPERMENT\data\joint_4_nndrc_Fld.mat  MatrixName=joint_4_nndrc_Fld
  To File39 : ToFile  Filename=C:\Users\ZJUCZ\Desktop\RBFNN_EXPERMENT\data\joint_4_nndrc_Qld.mat  MatrixName=joint_4_nndrc_Qld
  To File4 : ToFile  Commented=on  Filename=tracking_result_2  MatrixName=tracking_result
  To File40 : ToFile  Filename=C:\Users\ZJUCZ\Desktop\RBFNN_EXPERMENT\data\joint_3_nndrc_q.mat  MatrixName=joint_3_nndrc_q
  To File41 : ToFile  Filename=C:\Users\ZJUCZ\Desktop\RBFNN_EXPERMENT\data\joint_4_nndrc_q.mat  MatrixName=joint_4_nndrc_q
  To File42 : ToFile  Filename=C:\Users\ZJUCZ\Desktop\RBFNN_EXPERMENT\data\joint_3_nndrc_qddot.mat  MatrixName=joint_3_nndrc_qddot
  To File43 : ToFile  Filename=C:\Users\ZJUCZ\Desktop\RBFNN_EXPERMENT\data\joint_4_nndrc_qddot.mat  MatrixName=joint_4_nndrc_qddot
  To File44 : ToFile  Commented=on  Filename=C:\Users\ZJUCZ\Desktop\RBFNN_EXPERMENT\data\joint_3_drc_error.mat  MatrixName=joint_3_drc_error
  To File45 : ToFile  Commented=on  Filename=C:\Users\ZJUCZ\Desktop\RBFNN_EXPERMENT\data\joint_4_drc_error.mat  MatrixName=joint_4_drc_error
  To File46 : ToFile  Commented=on  Filename=C:\Users\ZJUCZ\Desktop\RBFNN_EXPERMENT\data\joint_3_drc_qd.mat  MatrixName=joint_3_drc_qd
  To File47 : ToFile  Commented=on  Filename=C:\Users\ZJUCZ\Desktop\RBFNN_EXPERMENT\data\joint_4_drc_qd.mat  MatrixName=joint_4_drc_qd
  To File48 : ToFile  Commented=on  Filename=C:\Users\ZJUCZ\Desktop\RBFNN_EXPERMENT\data\joint_4_drc_P_i.mat  MatrixName=joint_4_drc_P_i
  To File49 : ToFile  Commented=on  Filename=C:\Users\ZJUCZ\Desktop\RBFNN_EXPERMENT\data\joint_3_drc_P_i.mat  MatrixName=joint_3_drc_P_i
  To File5 : ToFile  Commented=on  Filename=theta_2  MatrixName=theta
  To File50 : ToFile  Commented=on  Filename=C:\Users\ZJUCZ\Desktop\RBFNN_EXPERMENT\data\joint_4_drc_P_o.mat  MatrixName=joint_4_drc_P_o
  To File51 : ToFile  Commented=on  Filename=C:\Users\ZJUCZ\Desktop\RBFNN_EXPERMENT\data\joint_3_drc_P_o.mat  MatrixName=joint_3_drc_P_o
  To File52 : ToFile  Commented=on  Filename=C:\Users\ZJUCZ\Desktop\RBFNN_EXPERMENT\data\joint_3_drc_U.mat  MatrixName=joint_3_drc_U
  To File53 : ToFile  Commented=on  Filename=C:\Users\ZJUCZ\Desktop\RBFNN_EXPERMENT\data\joint_4_drc_U.mat  MatrixName=joint_4_drc_U
  To File54 : ToFile  Commented=on  Filename=C:\Users\ZJUCZ\Desktop\RBFNN_EXPERMENT\data\joint_3_drc_Fld.mat  MatrixName=joint_3_drc_Fld
  To File55 : ToFile  Commented=on  Filename=C:\Users\ZJUCZ\Desktop\RBFNN_EXPERMENT\data\joint_3_drc_Qld.mat  MatrixName=joint_3_drc_Qld
  To File56 : ToFile  Commented=on  Filename=C:\Users\ZJUCZ\Desktop\RBFNN_EXPERMENT\data\joint_4_drc_Fld.mat  MatrixName=joint_4_drc_Fld
  To File57 : ToFile  Commented=on  Filename=C:\Users\ZJUCZ\Desktop\RBFNN_EXPERMENT\data\joint_4_drc_Qld.mat  MatrixName=joint_4_drc_Qld
  To File58 : ToFile  Commented=on  Filename=C:\Users\ZJUCZ\Desktop\RBFNN_EXPERMENT\data\joint_3_drc_q.mat  MatrixName=joint_3_drc_q
  To File59 : ToFile  Commented=on  Filename=C:\Users\ZJUCZ\Desktop\RBFNN_EXPERMENT\data\joint_4_drc_q.mat  MatrixName=joint_4_drc_q
  To File6 : ToFile  Commented=on  Filename=xv_2  MatrixName=xv
  To File60 : ToFile  Commented=on  Filename=C:\Users\ZJUCZ\Desktop\RBFNN_EXPERMENT\data\joint_3_drc_qddot.mat  MatrixName=joint_3_drc_qddot
  To File61 : ToFile  Commented=on  Filename=C:\Users\ZJUCZ\Desktop\RBFNN_EXPERMENT\data\joint_4_drc_qddot.mat  MatrixName=joint_4_drc_qddot
  To File62 : ToFile  Filename=C:\Users\ZJUCZ\Desktop\RBFNN_EXPERMENT\data\joint_3_nndrc_Fnn.mat  MatrixName=joint_3_nndrc_Fnn
  To File63 : ToFile  Filename=C:\Users\ZJUCZ\Desktop\RBFNN_EXPERMENT\data\joint_3_nndrc_Qnn.mat  MatrixName=joint_3_nndrc_Qnn
  To File66 : ToFile  Filename=C:\Users\ZJUCZ\Desktop\RBFNN_EXPERMENT\data\joint_4_nndrc_Fnn.mat  MatrixName=joint_4_nndrc_Fnn
  To File67 : ToFile  Filename=C:\Users\ZJUCZ\Desktop\RBFNN_EXPERMENT\data\joint_4_nndrc_Qnn.mat  MatrixName=joint_4_nndrc_Qnn
  To File7 : ToFile  Commented=on  Filename=p_2  MatrixName=p
  To File8 : ToFile  Commented=on  Filename=C:\Users\ZJUCZ\Desktop\RBFNN_EXPERMENT\joint4_e1  MatrixName=joint4_e1
  To File9 : ToFile  Commented=on  Filename=C:\Users\ZJUCZ\Desktop\RBFNN_EXPERMENT\joint4_e2  MatrixName=joint4_e2
  Unit Delay : UnitDelay  Commented=on  SampleTime=-1
  VS Communication (Visual Signal) : Subsystem  Commented=on
  bias{,1..3} (4 alike) : Sum  Commented=on  Inputs=++|
  break : Constant  Value=-1
  break1 : Constant
  close loop : Constant  Value=-1
  constant Velocity (m/s)1 : Constant  Commented=on  Value=0
  controller parameter1 : Subsystem  Commented=on
  controller parameter3 : Subsystem  Commented=on
  controller parameter4 : Subsystem  Commented=on
  controller parameter5 : Subsystem  Commented=on
  degree2rad{,1..3,9} (5 alike) : Gain  Commented=on  Gain=1/360*2*pi
  degree2rad10 : Gain  Gain=-1/360*2*pi
  degree2rad{4..8,11..12} (7 alike) : Gain  Gain=1/360*2*pi
  degree2rad13 : Gain  Gain=-1/360*2*pi
  dx_{1..4} (4 alike) : Scope  Commented=on  NumInputPorts=3
  e1_scope : Scope  NumInputPorts=4
  e2_scope : Scope  NumInputPorts=4
  e3_scope : Scope  NumInputPorts=4
  e=q-qd : Display
  g_d1 : Mux
  g_d2 : Mux
  gripper : ManualSwitch  CurrentSetting=0
  ini_bias : Constant  Commented=on  Value=0
  ini_bias1 : Constant  Commented=on  Value=10
  ini_bias2 : Constant  Commented=on  Value=60
  ini_bias3 : Constant  Commented=on  Value=0
  k_obs4 : Constant  Commented=on  Value=[1*10^2.5;5*10^4.2;2*10^6.3]  VectorParams1D=off
  limit_u : MATLAB Function  Commented=on  TreatAsAtomicUnit=on
  limit_u1 : MATLAB Function  Commented=on  TreatAsAtomicUnit=on
  limit_u2 : MATLAB Function  Commented=on  TreatAsAtomicUnit=on
  limit_u3 : MATLAB Function  Commented=on  TreatAsAtomicUnit=on
  look_e1 : Scope  NumInputPorts=4
  open loop : Constant  Value=0
  pin_pout : Scope  Commented=on  NumInputPorts=2
  pressure detect : Subsystem  Commented=on
  pressure detect1 : Subsystem  Commented=on
  pressure detect2 : Subsystem  Commented=on
  pressure detect3 : Subsystem  Commented=on
  q,qd,qdd,qddd{,1..3} (4 alike) : Mux  Commented=on
  q2qfdot_rad : MATLAB Function  TreatAsAtomicUnit=on
  qd{,1..3} (4 alike) : Scope  Commented=on  NumInputPorts=4
  "qd " : Display
  qd(°){,1..3} (4 alike) : Constant  Commented=on  Value=40
  qd(°){4..7} (4 alike) : Constant  Value=40
  qd_ddot{,1..3} (4 alike) : Constant  Commented=on  Value=20
  qd_ddot{4..7} (4 alike) : Constant  Value=30
  qd_dot{,1..3} (4 alike) : Constant  Commented=on  Value=20
  qd_dot{4..7} (4 alike) : Constant  Value=30
  qd_scope : Scope  NumInputPorts=4
  qr : Display
  rad2degree : Gain  Gain=2*pi/360
  run : Constant  Value=0
  run1 : Constant  Value=0
  t : Clock  Commented=on
  t1 : Clock
  theta{,1..3} (4 alike) : Scope  Commented=on  NumInputPorts=7
  "theta_s1_scope " : Scope  NumInputPorts=3
  "theta_s2_scope " : Scope  NumInputPorts=3
  ts : Constant  Commented=on  Value=0.001
  ts1 : Constant  Value=0.001
  u{,1..3} (4 alike) : Scope  Commented=on
  velocity caculator : Subsystem  Commented=on
  velocity caculator1 : Subsystem  Commented=on
  velocity caculator2 : Subsystem  Commented=on
  velocity caculator3 : Subsystem  Commented=on
  velocity caculator4 : Subsystem  Commented=on
  velocity caculator5 : Subsystem  Commented=on
  velocity caculator6 : Subsystem  Commented=on
  velocity caculator7 : Subsystem  Commented=on
  w2 : Mux
  w3 : Mux
  x{1..4} (4 alike) : Scope  Commented=on  NumInputPorts=2
  xv : Scope  Commented=on
  一键ARC : ManualSwitch
  置零{,1..3} (4 alike) : Constant  Commented=on
  wires:
  Bus Creator/1 -> x1/1
  Mux1/1 -> S-Function2/1
  Mux/1 -> Mux1/1
  velocity caculator/1(dxr) -> Manual Switch14/1, Sum3/2, dx_1/2
  pressure detect/1(pin) -> pin_pout/1, Mux5/1, Mux/3
  S-Function2/1 -> Demux/1
  Divide/1 -> Display3/1, limit_u/1(u), u/1
  Mux2/1 -> Switch2/3
  Mux7/1 -> Switch2/1
  Switch2/1 -> Mux1/2
  Constant1/1 -> Divide/2
  置零/1 -> Manual Switch3/1
  Constant6/1 -> Manual Switch3/2
  Constant7/1 -> Mux7/2, Mux7/4, Mux7/3
  From57/1 -> Gain10/1
  From/1 -> Gain9/1
  Demux/2 -> Mux6/2, theta/2
  Demux/4 -> Mux6/4, theta/4
  Demux/5 -> Mux6/5, theta/5
  Demux/6 -> Mux6/6, theta/6
  Demux/1 -> Mux6/1, theta/1
  Demux/8 -> Unit Delay/1
  Demux/18 -> Display6/1, Divide/1, xv/1
  pressure detect/2(pout) -> Mux5/2, pin_pout/2, Mux/4
  Mux5/1 -> Goto3/1
  Demux/3 -> Mux6/3, theta/3
  Demux/7 -> Mux6/7, theta/7
  Mux6/1 -> Goto7/1
  limit_u/1(y) -> Gain1/1
  From59/1 -> Gain11/1
  Mux8/1 -> Switch3/3
  Constant14/1 -> Mux9/2, Mux9/4, Mux9/3
  Mux9/1 -> Switch3/1
  From2/1 -> Gain8/1
  Bus Creator1/1 -> x2/1
  Mux10/1 -> Mux12/1
  Switch3/1 -> Mux12/2
  Mux12/1 -> S-Function1/1
  Demux1/2 -> Mux14/2, theta1/2
  S-Function1/1 -> Demux1/1
  Demux1/4 -> Mux14/4, theta1/4
  Mux14/1 -> Goto10/1
  Demux1/7 -> Mux14/7, theta1/7
  Demux1/3 -> Mux14/3, theta1/3
  Demux1/8 -> Goto23/1
  Demux1/1 -> Mux14/1, theta1/1
  Demux1/5 -> Mux14/5, theta1/5
  Demux1/6 -> Mux14/6, theta1/6
  Divide1/1 -> Display13/1, limit_u1/1(u), u1/1
  Constant16/1 -> Divide1/2
  Demux1/18 -> Display14/1, Divide1/1
  limit_u1/1(y) -> Gain4/1
  Mux15/1 -> Goto8/1
  pressure detect1/1(pin) -> Mux10/3, Scope/1, Mux15/1
  pressure detect1/2(pout) -> Mux15/2, Scope/2, Mux10/4
  Mux16/1 -> qr/1
  Angle from IMU/1(q1) -> Bias/1
  Angle from IMU/2(q2) -> Gain30/1
  Constant79/1 -> Nan Switch/2(angle signal)
  [control2] -> Mux17/2
  Mux17/1 -> Nan Switch/1(control input)
  [control1] -> Mux17/1
  Nan Switch/1(control) -> Demux2/1
  VS Communication (Visual Signal)/3(Error) -> Display19/1
  Gain10/1 -> Mux7/1, Switch/1
  Gain11/1 -> Switch1/1, Mux9/1
  Angle from IMU/3("q3 ") -> Bias1/1
  Angle from IMU/4(q4) -> Bias2/1
  Bias/1 -> Bias6/1
  Constant25/1 -> Switch5/1, Manual Switch11/1, Manual Switch8/1, Manual Switch4/1
  Constant30/1 -> Manual Switch5/1, Manual Switch12/1, Manual Switch13/1, Manual Switch9/1
  Switch9/1 -> Switch5/2
  Switch6/1 -> Manual Switch4/2
  [Control4] -> Switch9/3
  [Control3] -> Switch8/3
  [Control2] -> Switch7/3
  Manual Switch9/1 -> Switch7/1
  Manual Switch13/1 -> Switch8/1
  Switch7/1 -> Manual Switch8/2
  Manual Switch5/1 -> Switch6/1
  Bias12/1 -> HIL Write/2
  Gain12/1 -> Switch9/1
  Bias13/1 -> HIL Write/4
  [Switch_Val] -> Switch9/2, Switch8/2, Switch7/2, Switch6/2
  [Control1] -> Switch6/3
  Switch8/1 -> Manual Switch11/2
  Bias14/1 -> HIL Write/3
  Constant24/1 -> Manual Switch12/2, Manual Switch5/2, Manual Switch9/2, Manual Switch13/2
  Manual Switch12/1 -> Gain12/1
  close loop/1 -> CloseLoop/2
  CloseLoop/1 -> [Switch_Val]
  open loop/1 -> CloseLoop/1
  Unit Delay/1 -> Goto15/1
  From3/1 -> Subsystem/3(theta)
  Subsystem/1(Output) -> Demux9/1
  Demux9/5 -> Manual Switch7/2, Analog Filter Design3/1
  Sum3/1 -> dx_1/3
  Mux4/1 -> Goto17/1
  Gain2/1 -> Goto18/1
  Mux11/1 -> Goto19/1
  Gain5/1 -> Goto20/1
  From14/1 -> To File2/1
  From17/1 -> To File1/1
  From8/1 -> To File/1
  From19/1 -> To File3/1
  From22/1 -> To File4/1
  From21/1 -> To File7/1
  From20/1 -> To File5/1
  From23/1 -> To File6/1
  Obs Para Generator1/1(k_obs) -> Manual Switch2/1
  k_obs4/1 -> Manual Switch2/2
  Constant10/1 -> Obs Para Generator1/2(gain)
  Manual Switch2/1 -> Subsystem/4(k_obs)
  Constant9/1 -> Obs Para Generator1/1(a)
  Analog Filter Design3/1 -> Manual Switch7/1, Sum3/1, dx_1/1
  Constant17/1 -> Obs Para Generator1/3(th)
  From27/1 -> Mux/2
  Constant18/1 -> MATLAB Function/1(bias)
  MATLAB Function/1(out) -> Goto33/1
  Demux/28 -> Scope12/1
  Demux/29 -> Scope12/2
  From1/1 -> Subsystem/2(u)
  Gain9/1 -> Subsystem2/2(xr), Mux/1, velocity caculator/1(xr), Subsystem/1(xp), Display5/1
  Discrete PID Controller1/1 -> [PIDJ1]
  [PIDJ1] -> PID/ARC1/1, Display1/1
  Switch/1 -> Subsystem2/1(xd), Mux4/1, Bus Creator/1
  Subsystem2/1(qr) -> Goto74/1, Mux4/2, Bus Creator/2
  Subsystem2/2(e) -> x1/2, Goto80/1, Mux4/3
  Switch1/1 -> Mux11/1, Bus Creator1/1, Subsystem3/1(xd)
  Subsystem3/1(qr) -> Mux11/2, Bus Creator1/2, Goto76/1
  Sum1/1 -> dx_3/3
  velocity caculator1/1(dxr) -> dx_3/2, Sum1/2, Manual Switch10/2
  Obs Para Generator2/1(k_obs) -> Subsystem4/4(k_obs)
  Demux4/5 -> Analog Filter Design4/1
  From29/1 -> Subsystem4/2(u)
  Gain8/1 -> Subsystem3/2(xr), Mux10/1, Subsystem4/1(xp), velocity caculator1/1(xr)
  Manual Switch10/1 -> Goto26/1
  Analog Filter Design4/1 -> Manual Switch10/1, Sum1/1, dx_3/1
  From31/1 -> Subsystem4/3(theta)
  Subsystem4/1(Output) -> Demux4/1
  Constant2/1 -> Obs Para Generator2/2(gain)
  Constant19/1 -> Obs Para Generator2/1(a)
  Constant3/1 -> Obs Para Generator2/3(th)
  From11/1 -> Mux10/2
  From34/1 -> To File10/1
  From33/1 -> To File13/1
  From32/1 -> To File11/1
  From35/1 -> To File12/1
  Constant35/1 -> Obs Para Generator3/2(gain)
  Obs Para Generator3/1(k_obs) -> Subsystem5/4(k_obs)
  Subsystem1/2(e) -> Goto79/1, Gain18/1, Mux19/3
  Switch4/1 -> Mux19/1, Bus Creator2/1, Subsystem1/1(xd)
  Gain14/1 -> Goto29/1
  Subsystem1/1(qr) -> Mux19/2, Goto75/1, Bus Creator2/2
  Gain15/1 -> Subsystem1/2(xr), Mux13/1, Subsystem5/1(xp), velocity caculator2/1(xr)
  Divide2/1 -> Display12/1, limit_u2/1(u), u2/1
  velocity caculator2/1(dxr) -> dx_2/2, Sum5/2, Manual Switch15/2
  Demux3/8 -> Goto30/1
  Demux3/3 -> Mux22/3, theta2/3
  Mux19/1 -> Gain19/1
  Bus Creator2/1 -> Gain17/1
  Switch10/1 -> Mux20/2
  limit_u2/1(y) -> Gain13/1
  Demux3/1 -> Mux22/1, theta2/1
  Demux3/2 -> Mux22/2, theta2/2
  pressure detect2/2(pout) -> Mux23/2, Scope14/2, Mux13/4
  Constant34/1 -> Obs Para Generator3/1(a)
  pressure detect2/1(pin) -> Mux13/3, Scope14/1, Mux23/1
  Mux23/1 -> Goto32/1
  Demux3/18 -> Display16/1, Divide2/1
  From58/1 -> Gain3/1
  Gain13/1 -> Goto34/1, Display21/1, Scope20/1, Gain14/1
  Constant33/1 -> Divide2/2
  Demux3/6 -> Mux22/6, theta2/6
  Mux24/1 -> Switch10/3
  S-Function3/1 -> Demux3/1
  Demux3/4 -> Mux22/4, theta2/4
  Constant31/1 -> Mux25/2, Mux25/4, Mux25/3
  Mux22/1 -> Goto21/1
  Gain3/1 -> Switch4/1, Mux25/1
  From37/1 -> Gain15/1
  Mux20/1 -> S-Function3/1
  Constant36/1 -> Obs Para Generator3/3(th)
  Analog Filter Design5/1 -> dx_2/1, Manual Switch15/1, Sum5/1
  Demux3/5 -> Mux22/5, theta2/5
  Demux5/5 -> Analog Filter Design5/1
  Demux3/7 -> Mux22/7, theta2/7
  Mux13/1 -> Mux20/1
  From40/1 -> Subsystem5/3(theta)
  From38/1 -> Subsystem5/2(u)
  Mux25/1 -> Switch10/1
  Subsystem5/1(Output) -> Demux5/1
  Manual Switch15/1 -> Goto31/1
  Sum5/1 -> dx_2/3
  From36/1 -> Mux13/2
  Discrete PID Controller5/1 -> [pid2]
  Subsystem3/2(e) -> Goto81/1, x2/2, Mux11/3
  [arc1] -> PID/ARC1/2, Display23/1
  [pid2] -> PID/ARC2/1, Display8/1
  [arc2] -> Display25/1, PID/ARC2/2
  Gain4/1 -> Display18/1, MATLAB Function1/2(xv), Scope9/1, Gain5/1
  MATLAB Function1/1(out) -> Goto35/1
  Constant37/1 -> MATLAB Function1/1(bias)
  [pid3] -> Display26/1, PID/ARC3/1
  [arc3] -> Display27/1, PID/ARC3/2
  [temp2] -> Mux26/2
  [temp3] -> Mux26/3
  [temp1] -> Mux26/1
  [arc1] -> Mux27/1
  [pid2] -> Mux27/2
  [arc3] -> Mux27/3
  Demux6/1 -> [Control1]
  Demux6/2 -> [Control2]
  Demux6/3 -> [Control3]
  Mux26/1 -> 一键ARC/1
  Mux27/1 -> 一键ARC/2
  Demux6/4 -> [Control4]
  [temp4] -> Mux26/4
  [arc4] -> Mux27/4
  From50/1 -> Switch/2, Switch2/2
  Manual Switch3/1 -> Goto40/1
  Constant5/1 -> Manual Switch18/2
  置零2/1 -> Manual Switch18/1
  Manual Switch18/1 -> Goto41/1
  Manual Switch19/1 -> Goto42/1
  置零3/1 -> Manual Switch19/1
  Constant39/1 -> Manual Switch19/2
  From51/1 -> Switch10/2, Switch4/2
  From52/1 -> Switch3/2, Switch1/2
  Mux28/1 -> "qd "/1
  [qd1] -> Gain/1
  [qd3] -> Gain16/1
  [qd2] -> Gain6/1
  Gain/1 -> qd_scope/1, Add1/2, Mux28/1
  Gain16/1 -> qd_scope/3, Add3/2, Mux28/3
  [qd4] -> Gain23/1
  17.73/1 -> Goto47/1
  -25/1 -> Goto48/1
  89.3/1 -> Goto49/1
  controller parameter3/9(gam6) -> Mux29/9
  controller parameter3/6(gam3) -> Mux29/6
  controller parameter3/11(gam8) -> Mux29/11
  controller parameter3/8(gam5) -> Mux29/8
  Mux29/1 -> Goto50/1
  controller parameter3/10(gam7) -> Mux29/10
  controller parameter3/4(gam1) -> Mux29/4
  controller parameter3/3(k3) -> Mux29/3
  controller parameter3/2(k2) -> Mux29/2
  controller parameter3/7(gam4) -> Mux29/7
  controller parameter3/5(gam2) -> Mux29/5
  controller parameter3/1(k1) -> Mux29/1
  From60/1 -> Mux1/3
  Mux3/1 -> Goto51/1
  controller parameter4/1(k1) -> Mux3/1
  controller parameter4/7(gam4) -> Mux3/7
  controller parameter4/5(gam2) -> Mux3/5
  controller parameter4/3(k3) -> Mux3/3
  controller parameter4/2(k2) -> Mux3/2
  controller parameter4/4(gam1) -> Mux3/4
  controller parameter4/10(gam7) -> Mux3/10
  controller parameter4/6(gam3) -> Mux3/6
  controller parameter4/11(gam8) -> Mux3/11
  controller parameter4/9(gam6) -> Mux3/9
  controller parameter4/8(gam5) -> Mux3/8
  controller parameter5/9(gam6) -> Mux30/9
  controller parameter5/8(gam5) -> Mux30/8
  controller parameter5/7(gam4) -> Mux30/7
  controller parameter5/4(gam1) -> Mux30/4
  controller parameter5/6(gam3) -> Mux30/6
  controller parameter5/11(gam8) -> Mux30/11
  controller parameter5/2(k2) -> Mux30/2
  controller parameter5/10(gam7) -> Mux30/10
  controller parameter5/3(k3) -> Mux30/3
  Mux30/1 -> Goto52/1
  controller parameter5/5(gam2) -> Mux30/5
  controller parameter5/1(k1) -> Mux30/1
  From61/1 -> Mux20/3
  From62/1 -> Mux12/3
  Gain17/1 -> x3/1
  Gain18/1 -> x3/2
  Gain19/1 -> Goto28/1
  Mux21/1 -> Goto54/1
  Demux7/8 -> Goto56/1
  Gain20/1 -> Goto59/1, Display31/1, Scope15/1, Gain21/1
  From64/1 -> Gain22/1
  From69/1 -> Mux31/3
  S-Function4/1 -> Demux7/1
  Analog Filter Design7/1 -> Manual Switch1/1, Sum6/1, dx_4/1
  limit_u3/1(y) -> Gain20/1
  Demux8/5 -> Analog Filter Design7/1
  Mux18/1 -> Mux31/1
  From67/1 -> Switch12/2, Switch13/2
  Switch12/1 -> Mux31/2
  Mux35/1 -> Switch12/1
  Mux34/1 -> Switch12/3
  pressure detect3/1(pin) -> Mux18/3, Scope4/1, Mux33/1
  Demux7/5 -> Mux32/5, theta3/5
  Bus Creator3/1 -> x4/1
  Demux7/1 -> Mux32/1, theta3/1
  velocity caculator3/1(dxr) -> dx_4/2, Sum6/2, Manual Switch1/2
  Demux7/6 -> Mux32/6, theta3/6
  Obs Para Generator4/1(k_obs) -> Subsystem7/4(k_obs)
  Mux31/1 -> S-Function4/1
  From63/1 -> Mux18/2
  Subsystem7/1(Output) -> Demux8/1
  Divide3/1 -> Display28/1, limit_u3/1(u), u3/1
  Sum6/1 -> dx_4/3
  Demux7/7 -> Mux32/7, theta3/7
  Manual Switch1/1 -> Goto57/1
  From66/1 -> Subsystem7/3(theta)
  Demux7/4 -> Mux32/4, theta3/4
  Constant11/1 -> Mux35/2, Mux35/4, Mux35/3
  Constant23/1 -> Divide3/2
  From68/1 -> Gain26/1
  Demux7/3 -> Mux32/3, theta3/3
  Demux7/2 -> Mux32/2, theta3/2
  pressure detect3/2(pout) -> Mux33/2, Scope4/2, Mux18/4
  From65/1 -> Subsystem7/2(u)
  Mux33/1 -> Goto58/1
  Gain26/1 -> Switch13/1, Mux35/1
  Constant40/1 -> Obs Para Generator4/1(a)
  Mux32/1 -> Goto53/1
  Subsystem6/1(qr) -> Goto77/1, Bus Creator3/2, Mux21/2
  Demux7/18 -> Display29/1, Divide3/1
  Gain21/1 -> Goto55/1
  Switch13/1 -> Mux21/1, Bus Creator3/1, Subsystem6/1(xd)
  Constant42/1 -> Obs Para Generator4/3(th)
  Constant41/1 -> Obs Para Generator4/2(gain)
  Gain22/1 -> Subsystem6/2(xr), Mux18/1, Subsystem7/1(xp), velocity caculator3/1(xr)
  24.22/1 -> Goto63/1
  Manual Switch6/1 -> Goto62/1
  置零1/1 -> Manual Switch6/1
  [arc4] -> Display33/1, PID/ARC4/2
  [pid4] -> Display32/1, PID/ARC4/1
  Constant44/1 -> Manual Switch6/2
  Demux2/1 -> [temp1]
  Demux2/2 -> [temp2]
  Demux2/3 -> [temp3]
  Demux2/4 -> [temp4]
  PID/ARC1/1 -> [control1]
  PID/ARC4/1 -> [control4]
  PID/ARC3/1 -> [control3]
  PID/ARC2/1 -> [control2]
  [control3] -> Mux17/3
  [control4] -> Mux17/4
  From74/1 -> To File16/1
  From76/1 -> To File15/1
  From75/1 -> To File18/1
  From77/1 -> To File17/1
  controller parameter1/1(k1) -> Mux36/1
  Mux36/1 -> Goto67/1
  controller parameter1/5(gam2) -> Mux36/5
  controller parameter1/10(gam7) -> Mux36/10
  controller parameter1/6(gam3) -> Mux36/6
  controller parameter1/7(gam4) -> Mux36/7
  controller parameter1/11(gam8) -> Mux36/11
  controller parameter1/4(gam1) -> Mux36/4
  controller parameter1/8(gam5) -> Mux36/8
  controller parameter1/9(gam6) -> Mux36/9
  controller parameter1/3(k3) -> Mux36/3
  controller parameter1/2(k2) -> Mux36/2
  Gain23/1 -> qd_scope/4, Add4/2, Mux28/4
  constant Velocity (m/s)1/1 -> Subsystem8/1(In1)
  Subsystem8/1(xyz) -> Demux14/1
  Demux14/1 -> Scope10/1
  Demux14/2 -> Scope10/2
  Demux14/3 -> Scope10/3
  Subsystem8/6(J5) -> Display24/1, Goto5/1
  Constant4/1 -> Goto71/1
  From86/1 -> To File20/1
  From82/1 -> To File21/1
  Demux17/1 -> Goto60/1, Mux34/1, Switch13/3
  velocity caculator/2(dxb) -> Manual Switch14/2
  Manual Switch16/1 -> Delay/1
  Manual Switch7/1 -> Manual Switch16/1
  Manual Switch14/1 -> Manual Switch16/2
  Delay/1 -> Goto16/1
  Demux11/1 -> Goto43/1, Switch/3, Mux2/1
  Gain1/1 -> Scope8/1, Gain2/1, MATLAB Function/2(xv), Display17/1
  Demux12/1 -> Goto44/1, Mux8/1, Switch1/3
  Demux13/1 -> Goto45/1, Mux24/1, Switch4/3
  [e2] -> degree2rad11/1
  [e3] -> degree2rad12/1
  Discrete PID Controller3/1 -> [pid3]
  Subsystem6/2(e) -> Goto82/1, x4/2, Mux21/3
  [e4] -> degree2rad13/1
  Discrete PID Controller2/1 -> [pid4]
  一键ARC/1 -> Demux6/1
  break/1 -> Break/2
  Break/1 -> Switch11/2
  run/1 -> Break/1
  Constant38/1 -> Switch11/3
  Manual Switch4/1 -> Mux37/1
  Switch5/1 -> Mux37/4
  Manual Switch11/1 -> Mux37/3
  Manual Switch8/1 -> Mux37/2
  Mux37/1 -> Switch11/1
  Switch11/1 -> Demux10/1
  Demux15/2 -> Scope11/2
  Subsystem9/6(Out6) -> Goto72/1, Display34/1
  Demux15/1 -> Scope11/1
  Subsystem9/4(Out4) -> Gain28/1
  Subsystem9/3(Out3) -> Gain27/1
  Subsystem9/1(Out1) -> Gain24/1
  Gain29/1 -> Subsystem9/1(In1)
  Gain25/1 -> Goto68/1
  Subsystem9/7(Out7) -> Demux16/1, Goto73/1
  Demux16/1 -> Scope16/1
  From88/1 -> Mux38/2
  Demux16/2 -> Scope16/2
  Constant/1 -> Manual Switch/1
  From89/1 -> Mux38/3
  Manual Switch/1 -> Subsystem9/2(reset)
  Gain28/1 -> Goto70/1
  Mux38/1 -> Gain29/1
  Subsystem9/5(Out5) -> Goto78/1, Demux15/1
  Demux16/3 -> Scope16/3
  Demux15/3 -> Scope11/3
  From87/1 -> Mux38/4
  Constant13/1 -> Manual Switch/2
  Subsystem9/2(Out2) -> Gain25/1
  Gain27/1 -> Goto69/1
  From90/1 -> Mux38/1
  Gain24/1 -> Goto/1
  From83/1 -> Demux11/1
  Demux11/2 -> Mux2/2
  Demux11/3 -> Mux2/3
  Demux11/4 -> Mux2/4
  From84/1 -> Demux13/1
  Demux13/2 -> Mux24/2
  Demux13/3 -> Mux24/3
  Demux13/4 -> Mux24/4
  From85/1 -> Demux12/1
  Demux12/2 -> Mux8/2
  Demux12/3 -> Mux8/3
  Demux12/4 -> Mux8/4
  From91/1 -> Demux17/1
  Demux17/2 -> Mux34/2
  Demux17/3 -> Mux34/3
  Demux17/4 -> Mux34/4
  MATLAB Function10/3(a) -> " 4"/1
  "  4"/1 -> Goto83/1
  qd_ddot3/1 -> MATLAB Function10/3(a_max)
  q,qd,qdd,qddd/1 -> Goto24/1
  t/1 -> MATLAB Function9/5(t), MATLAB Function10/5(t), MATLAB Function8/5(t), MATLAB Function7/5(t)
  ini_bias1/1 -> bias1/1
  "   3"/1 -> qd3/2, q,qd,qdd,qddd3/2
  MATLAB Function9/1(s) -> bias2/2
  qd(°)3/1 -> MATLAB Function10/1(p_end)
  q,qd,qdd,qddd2/1 -> "  5"/1
  MATLAB Function9/2(v) -> "   2"/1
  q,qd,qdd,qddd3/1 -> Goto88/1
  MATLAB Function10/2(v) -> "   3"/1
  " 2"/1 -> q,qd,qdd,qddd1/3, qd1/3
  bias3/1 -> degree2rad3/1
  "   1"/1 -> qd1/2, q,qd,qdd,qddd1/2
  "   2"/1 -> qd2/2, q,qd,qdd,qddd2/2
  "   "/1 -> qd/2, q,qd,qdd,qddd/2
  degree2rad1/1 -> qd1/1, q,qd,qdd,qddd1/1
  bias/1 -> degree2rad/1
  MATLAB Function10/1(s) -> bias3/2
  MATLAB Function8/1(s) -> bias1/2
  degree2rad2/1 -> qd2/1, q,qd,qdd,qddd2/1
  degree2rad/1 -> qd/1, q,qd,qdd,qddd/1
  " 3"/1 -> q,qd,qdd,qddd2/3, qd2/3
  bias1/1 -> degree2rad1/1
  "  5"/1 -> Goto87/1
  MATLAB Function9/3(a) -> " 3"/1
  MATLAB Function8/3(a) -> " 2"/1
  MATLAB Function9/4(j) -> "  2"/1
  qd_dot3/1 -> MATLAB Function10/2(v_max)
  ini_bias3/1 -> bias3/1
  ini_bias2/1 -> bias2/1
  MATLAB Function7/4(j) -> "  "/1
  "  1"/1 -> q,qd,qdd,qddd1/4, qd1/4
  ts/1 -> MATLAB Function7/4(ts), MATLAB Function8/4(ts), MATLAB Function9/4(ts), MATLAB Function10/4(ts)
  bias2/1 -> degree2rad2/1
  qd_ddot2/1 -> MATLAB Function9/3(a_max)
  qd_dot1/1 -> MATLAB Function8/2(v_max)
  q,qd,qdd,qddd1/1 -> "  4"/1
  "  3"/1 -> q,qd,qdd,qddd3/4, qd3/4
  qd(°)1/1 -> MATLAB Function8/1(p_end)
  MATLAB Function8/2(v) -> "   1"/1
  qd_ddot1/1 -> MATLAB Function8/3(a_max)
  MATLAB Function10/4(j) -> "  3"/1
  qd(°)/1 -> MATLAB Function7/1(p_end)
  MATLAB Function7/3(a) -> " 1"/1
  "  "/1 -> q,qd,qdd,qddd/4, qd/4
  "  2"/1 -> q,qd,qdd,qddd2/4, qd2/4
  ini_bias/1 -> bias/1
  " 1"/1 -> q,qd,qdd,qddd/3, qd/3
  " 4"/1 -> q,qd,qdd,qddd3/3, qd3/3
  MATLAB Function7/2(v) -> "   "/1
  degree2rad3/1 -> qd3/1, q,qd,qdd,qddd3/1
  MATLAB Function7/1(s) -> bias/2
  qd_dot/1 -> MATLAB Function7/2(v_max)
  MATLAB Function8/4(j) -> "  1"/1
  qd_dot2/1 -> MATLAB Function9/2(v_max)
  qd_ddot/1 -> MATLAB Function7/3(a_max)
  qd(°)2/1 -> MATLAB Function9/1(p_end)
  DIARC_new/16(tolook_others) -> Demux24/1
  [Ps] -> DIARC_new/12(P_s)
  DIARC_new/4(vartheta_s1_next) -> Delay1/1
  Manual Switch20/1 -> DIARC_new/1(mode_IARC)
  Demux25/2 -> Scope13/2
  Demux20/12 -> Mux46/4
  Constant58/1 -> g_d2/2
  DIARC_new/13(X1f_next) -> Delay11/1
  Demux20/3 -> Mux44/3
  Demux25/1 -> Scope13/1
  Demux20/7 -> Mux45/3
  K_1/1 -> DIARC_new/14(K_1)
  Demux22/1 -> Mux51/1
  Mux55/1 -> Mux68/2
  Demux23/3 -> Mux41/3
  Demux23/7 -> Mux42/3
  Demux22/9 -> Mux51/3
  Demux23/1 -> Mux41/1
  Delay7/1 -> DIARC_new/26(Gamma1_2)
  Demux20/11 -> Mux46/3
  w3/1 -> DIARC_new/18(w3)
  Demux21/1 -> Mux47/1
  Demux23/2 -> Mux41/2
  Mux53/1 -> Mux66/2
  Demux23/5 -> Mux42/1
  DIARC_new/10(Gamma1_3_next) -> Delay8/1
  Demux23/8 -> Mux42/4
  Demux23/4 -> Mux41/4
  Demux22/4 -> Mux55/1
  Delay6/1 -> DIARC_new/25(Gamma1_1), Scope7/1
  [q] -> DIARC_new/8(q)
  Demux18/3 -> e2_scope/3
  Demux22/5 -> Mux51/2
  Demux23/9 -> "theta_s2_scope "/3
  Demux21/10 -> Mux48/3
  Constant57/1 -> g_d2/4
  Mux41/1 -> "theta_s2_scope "/1
  Mux42/1 -> "theta_s2_scope "/2
  Demux23/6 -> Mux42/2
  [P_i] -> DIARC_new/10(P_i)
  Demux22/10 -> Mux52/3
  Demux22/14 -> Mux52/4
  Demux21/3 -> Mux49/1
  Demux22/16 -> Mux55/4
  Demux22/15 -> Mux53/4
  Demux22/13 -> Mux51/4
  Constant65/1 -> K_1/2
  Demux22/11 -> Mux53/3
  DIARC_new/14(tolook_FLd) -> Demux21/1
  Demux22/3 -> Mux53/1
  Demux22/2 -> Mux52/1
  Demux22/8 -> Mux55/2
  Constant67/1 -> K_1/3
  Demux21/8 -> Mux50/2
  Constant68/1 -> K_1/4
  Constant61/1 -> g_d1/2
  [P_o] -> DIARC_new/11(P_o)
  DIARC_new/15(tolook_QLd) -> Demux22/1
  Constant32/1 -> K_3/2
  Demux18/1 -> e2_scope/1
  Constant20/1 -> K_2/4
  DIARC_new/2(e2) -> [z2], Demux18/1
  Demux21/5 -> Mux47/2
  Demux21/12 -> Mux50/3
  DIARC_new/7(d2hat_next) -> Delay5/1
  DIARC_new/11(Gamma1_4_next) -> Delay9/1
  DIARC_new/6(d1hat_next) -> Delay4/1
  Demux21/9 -> Mux47/3
  Mux49/1 -> Mux65/2
  Demux22/12 -> Mux55/3
  Mux50/1 -> Mux67/2
  Demux22/7 -> Mux53/2
  Demux19/1 -> e3_scope/1
  Constant64/1 -> Manual Switch20/2
  Constant53/1 -> w2/1
  Constant63/1 -> Manual Switch20/1
  Mux46/1 -> "theta_s1_scope "/3
  Demux20/10 -> Mux46/2
  Demux21/7 -> Mux49/2
  Mux45/1 -> "theta_s1_scope "/2
  Demux20/5 -> Mux45/1
  Mux44/1 -> "theta_s1_scope "/1
  Demux21/2 -> Mux48/1
  Demux20/4 -> Mux44/4
  Demux21/4 -> Mux50/1
  Demux21/6 -> Mux48/2
  Demux20/6 -> Mux45/2
  Mux48/1 -> Mux63/2
  DIARC_new/3(e3) -> [z3], Demux19/1
  Demux22/6 -> Mux52/2
  Demux19/2 -> e3_scope/2
  Constant47/1 -> w3/3
  Delay5/1 -> DIARC_new/24(d2hat)
  Demux20/8 -> Mux45/4
  w2/1 -> DIARC_new/17(w2)
  Demux19/3 -> e3_scope/3
  Demux18/2 -> e2_scope/2
  Constant48/1 -> w3/4
  Demux18/4 -> e2_scope/4
  DIARC_new/12(Gamma2_next) -> Delay13/1
  Delay11/1 -> DIARC_new/30(X1_f)
  [qd3_ddot] -> Mux43/3
  Mux40/1 -> DIARC_new/5(qd_dot)
  [qd1_ddot] -> Mux43/1
  Demux21/11 -> Mux49/3
  [qd2_ddot] -> Mux43/2
  Mux43/1 -> DIARC_new/6(qd_ddot)
  Constant45/1 -> w2/3
  Delay1/1 -> DIARC_new/21(vartheta_s1), Demux20/1
  [qd1_dot] -> Mux40/1
  Demux20/1 -> Mux44/1
  Constant59/1 -> g_d2/1
  Constant69/1 -> K_2/2
  [qd3] -> Mux39/3
  [qd1_dddot] -> Mux54/1
  [qd1] -> Mux39/1
  Constant43/1 -> K_3/1
  Demux20/2 -> Mux44/2
  [qd4_dot] -> Mux40/4
  Constant21/1 -> K_3/3
  K_2/1 -> DIARC_new/15(K_2)
  Constant15/1 -> K_2/3
  Constant22/1 -> K_3/4
  [qd4] -> Mux39/4
  Constant66/1 -> K_1/1
  Constant60/1 -> DIARC_new/13(P_r)
  Demux19/4 -> e3_scope/4
  K_3/1 -> DIARC_new/16(K_3)
  Constant51/1 -> w3/1
  Demux20/9 -> Mux46/1
  DIARC_new/1(U) -> Demux26/1, Demux25/1
  [q_dot] -> DIARC_new/9(q_dot)
  [qd3_dddot] -> Mux54/3
  Constant56/1 -> g_d2/3
  Constant54/1 -> g_d1/3
  Multiply1/1 -> DIARC_new/19(gamma_d1)
  Demux25/4 -> Scope13/4
  Constant62/1 -> g_d1/1
  Mux39/1 -> DIARC_new/4(qd)
  Delay4/1 -> DIARC_new/23(d1hat)
  [qd4_dddot] -> Mux54/4
  Constant55/1 -> g_d1/4
  [qd2] -> Mux39/2
  Multiply/1 -> DIARC_new/20(gamma_d2)
  Constant70/1 -> K_2/1
  [qd3_dot] -> Mux40/3
  DIARC_new/5(vartheta_s2_next) -> Delay2/1
  [qd2_dddot] -> Mux54/2
  [qd2_dot] -> Mux40/2
  Mux47/1 -> Mux60/2
  Delay2/1 -> Demux23/1, DIARC_new/22(vartheta_s2)
  DIARC_new/8(Gamma1_1_next) -> Delay6/1
  DIARC_new/9(Gamma1_2_next) -> Delay7/1
  Mux54/1 -> DIARC_new/7(qd_dddot)
  Constant52/1 -> w2/2
  Demux25/3 -> Scope13/3
  Constant46/1 -> w2/4
  Delay13/1 -> DIARC_new/29(Gamma2)
  Delay9/1 -> DIARC_new/28(Gamma1_4)
  [qd4_ddot] -> Mux43/4
  Delay8/1 -> DIARC_new/27(Gamma1_3)
  Constant50/1 -> w3/2
  "   7"/1 -> Product2/2
  J2_P2P(the out is degree°)/1(s) -> degree2rad5/1
  degree2rad6/1 -> Product7/2
  qd_dot7/1 -> J4_P2P(the out is degree°)/2(v_max)
  "   5"/1 -> Product10/2
  Product/1 -> [qd4_dddot]
  Product1/1 -> [qd4_ddot]
  qd(°)4/1 -> J1_P2P(the out is degree°)/1(p_end)
  Product4/1 -> [qd3_dddot]
  "  7"/1 -> Product8/2
  Product14/1 -> [qd1_dot]
  Product15/1 -> Bias7/1
  J4_P2P(the out is degree°)/1(s) -> degree2rad7/1
  Product5/1 -> [qd3_ddot]
  Product6/1 -> [qd3_dot]
  " "/1 -> Product13/2
  Manual Switch23/1 -> Product7/1, Product4/1, Product5/1, Product6/1
  " 7"/1 -> Product1/2
  Manual Switch24/1 -> Product3/1, Product/1, Product1/1, Product2/1
  Product12/1 -> [qd1_dddot]
  degree2rad4/1 -> Product15/2
  Product2/1 -> [qd4_dot]
  Manual Switch21/1 -> Product12/1, Product13/1, Product14/1, Product15/1
  Product13/1 -> [qd1_ddot]
  Product10/1 -> [qd2_dot]
  " 5"/1 -> Product9/2
  degree2rad5/1 -> Product11/2
  "   6"/1 -> Product6/2
  "  9"/1 -> Product/2
  qd(°)5/1 -> J2_P2P(the out is degree°)/1(p_end)
  J2_P2P(the out is degree°)/3(a) -> " 5"/1
  Constant72/1 -> Manual Switch21/2, Manual Switch22/2, Manual Switch24/2, Manual Switch23/2
  J1_P2P(the out is degree°)/3(a) -> " "/1
  J1_P2P(the out is degree°)/4(j) -> "  6"/1
  J3_P2P(the out is degree°)/4(j) -> "  8"/1
  Product3/1 -> Bias10/1
  qd_dot4/1 -> J1_P2P(the out is degree°)/2(v_max)
  " 6"/1 -> Product5/2
  J1_P2P(the out is degree°)/1(s) -> degree2rad4/1
  J2_P2P(the out is degree°)/2(v) -> "   5"/1
  "   4"/1 -> Product14/2
  J1_P2P(the out is degree°)/2(v) -> "   4"/1
  Product8/1 -> [qd2_dddot]
  qd_ddot7/1 -> J4_P2P(the out is degree°)/3(a_max)
  qd_ddot4/1 -> J1_P2P(the out is degree°)/3(a_max)
  Constant71/1 -> Manual Switch24/1, Manual Switch23/1, Manual Switch22/1, Manual Switch21/1
  degree2rad7/1 -> Product3/2
  J3_P2P(the out is degree°)/2(v) -> "   6"/1
  qd(°)6/1 -> J3_P2P(the out is degree°)/1(p_end)
  J4_P2P(the out is degree°)/2(v) -> "   7"/1
  J4_P2P(the out is degree°)/3(a) -> " 7"/1
  qd_dot6/1 -> J3_P2P(the out is degree°)/2(v_max)
  Product9/1 -> [qd2_ddot]
  qd(°)7/1 -> J4_P2P(the out is degree°)/1(p_end)
  ts1/1 -> q2qfdot_rad/1(ts), J4_P2P(the out is degree°)/4(ts), J3_P2P(the out is degree°)/4(ts), J2_P2P(the out is degree°)/4(ts), J1_P2P(the out is degree°)/4(ts)
  "  6"/1 -> Product12/2
  J3_P2P(the out is degree°)/1(s) -> degree2rad6/1
  qd_ddot6/1 -> J3_P2P(the out is degree°)/3(a_max)
  J3_P2P(the out is degree°)/3(a) -> " 6"/1
  qd_dot5/1 -> J2_P2P(the out is degree°)/2(v_max)
  Product11/1 -> Bias8/1
  J4_P2P(the out is degree°)/4(j) -> "  9"/1
  J2_P2P(the out is degree°)/4(j) -> "  7"/1
  "  8"/1 -> Product4/2
  qd_ddot5/1 -> J2_P2P(the out is degree°)/3(a_max)
  Manual Switch22/1 -> Product8/1, Product9/1, Product10/1, Product11/1
  Product7/1 -> Bias9/1
  t1/1 -> [time], J4_P2P(the out is degree°)/5(t), J3_P2P(the out is degree°)/5(t), J2_P2P(the out is degree°)/5(t), J1_P2P(the out is degree°)/5(t)
  P1/1(pin) -> Mux69/1, Mux56/1
  P2/2(pin) -> Mux70/1, Mux56/2
  P3/1(pin) -> Mux56/3, Mux71/1
  P4/1(pin) -> Mux56/4, Mux72/1
  P2/1(pout) -> Mux70/2, Mux57/2
  P3/2(pout) -> Mux57/3, Mux71/2
  P4/2(pout) -> Mux72/2, Mux57/4
  Mux56/1 -> MPa2Pa/1
  Mux57/1 -> MPa2Pa1/1
  [q1] -> Mux58/1
  [q2] -> Mux58/2
  [q3] -> Mux58/3
  [q4] -> Mux58/4
  Mux58/1 -> degree2rad8/1
  degree2rad8/1 -> [q]
  From107/1 -> velocity caculator4/1(xr)
  From108/1 -> velocity caculator5/1(xr)
  From109/1 -> velocity caculator6/1(xr)
  From110/1 -> velocity caculator7/1(xr)
  velocity caculator5/1(dxr) -> Mux59/2
  velocity caculator4/1(dxr) -> Mux59/1
  velocity caculator6/1(dxr) -> Mux59/3
  velocity caculator7/1(dxr) -> Mux59/4
  Mux59/1 -> degree2rad9/1
  degree2rad9/1 -> Goto106/1
  Demux26/4 -> [arc4]
  Demux26/1 -> [arc1]
  Demux26/2 -> [arc2]
  Demux26/3 -> [arc3]
  Constant80/1 -> DIARC_new/31(q_ddot)
  Gain30/1 -> Bias3/1
  Bias1/1 -> Gain31/1
  Gain31/1 -> Bias4/1
  Bias2/1 -> Gain32/1
  Gain32/1 -> Bias5/1
  Bias3/1 -> Mux16/2, Add2/1, [q2]
  Bias4/1 -> Add3/1, [q3], Mux16/3
  Bias5/1 -> Mux16/4, Add4/1, [q4]
  Mux61/1 -> e=q-qd/1, [z1]
  Add2/1 -> Mux61/2, e1_scope/2, [e2]
  Add3/1 -> Mux61/3, e1_scope/3, [e3]
  Add4/1 -> Mux61/4, e1_scope/4, [e4]
  Add1/1 -> Mux61/1, e1_scope/1, [e1]
  Gain6/1 -> qd_scope/2, Add2/2, Mux28/2
  Bias6/1 -> Add1/1, [q1], Mux16/1
  Demux10/1 -> Bias11/1
  Bias11/1 -> HIL Write/1
  Demux10/2 -> Bias12/1
  Demux10/3 -> Bias14/1
  Demux10/4 -> Bias13/1
  [e1] -> degree2rad10/1
  degree2rad10/1 -> Discrete PID Controller1/1
  degree2rad11/1 -> Discrete PID Controller5/1
  degree2rad12/1 -> Discrete PID Controller3/1
  degree2rad13/1 -> Discrete PID Controller2/1
  [qd4] -> Gain7/1
  [e4] -> Look_J4/2
  [e1] -> Look_J1/2
  Mux77/1 -> Look_J1/1
  [qd1] -> Gain33/1
  Mux51/1 -> Mux62/2
  [qd2] -> Gain34/1
  Mux78/1 -> Look_J2/1
  [e2] -> Look_J2/2
  [qd3] -> Gain35/1
  Mux79/1 -> Look_J3/1
  [e3] -> Look_J3/2
  Mux52/1 -> Mux64/2
  Demux24/1 -> Mux60/1
  Mux60/1 -> Look_J1/3
  Demux24/5 -> Mux62/1
  Mux62/1 -> Look_J1/4
  Demux24/2 -> Mux63/1
  Demux24/6 -> Mux64/1
  Mux64/1 -> Look_J2/4
  Mux63/1 -> Look_J2/3
  Demux24/3 -> [joint3_Fld], Mux65/1
  Demux24/7 -> Mux66/1, [joint3_Qld]
  Demux24/4 -> [joint4_Fld], Mux67/1
  Demux24/8 -> [joint4_Qld], Mux68/1
  Mux66/1 -> Look_J3/4
  Mux65/1 -> Look_J3/3
  Mux67/1 -> Look_J4/3
  Mux68/1 -> Look_J4/4
  Demux24/9 -> Scope1/1
  Demux24/10 -> Scope1/2
  Demux24/11 -> Scope1/3
  Demux24/12 -> Scope1/4
  Bias7/1 -> Add/2
  Add/1 -> [qd1]
  1/1 -> Add/1
  Constant26/1 -> 1/1
  2/1 -> Add5/1
  Constant27/1 -> 2/1
  Bias8/1 -> Add5/2
  Add5/1 -> [qd2]
  3/1 -> Add6/1
  Constant28/1 -> 3/1
  Bias9/1 -> Add6/2
  Add6/1 -> [qd3]
  4/1 -> Add7/1
  Constant29/1 -> 4/1
  Bias10/1 -> Add7/2
  Add7/1 -> [qd4]
  HIL Read Analog/1 -> MPa2Pa2/1
  Mux69/1 -> P_scope1/1
  Mux70/1 -> P_scope1/2
  Mux71/1 -> P_scope1/3
  Mux72/1 -> P_scope1/4
  P1/2(pout) -> Mux69/2, Mux57/1
  MPa2Pa/1 -> [P_i]
  MPa2Pa1/1 -> [P_o]
  MPa2Pa2/1 -> P_scope2/1, [Ps]
  [q] -> Demux27/1
  [q_dot] -> Demux28/1
  Mux73/1 -> Look_q qdot/1
  Demux27/1 -> Mux73/1
  Demux28/1 -> Mux73/2
  Mux74/1 -> Look_q qdot/2
  Demux27/2 -> Mux74/1
  Demux28/2 -> Mux74/2
  Mux76/1 -> Look_q qdot/4
  Mux75/1 -> Look_q qdot/3
  Demux27/3 -> Mux75/1
  Demux27/4 -> Mux76/1
  Demux28/3 -> Mux75/2
  Demux28/4 -> Mux76/2
  Demux24/13 -> look_e1/1
  Demux24/14 -> look_e1/2
  Demux24/15 -> look_e1/3
  Demux24/16 -> look_e1/4
  [qd4_dot] -> Mux76/3
  [qd3_dot] -> Mux75/3
  [qd2_dot] -> Mux74/3
  [qd1_dot] -> Mux73/3
  Gain33/1 -> Mux77/2
  [q1] -> Mux77/1
  Gain34/1 -> Mux78/2
  [q2] -> Mux78/1
  Gain35/1 -> Mux79/2
  [q3] -> Mux79/1
  Mux80/1 -> Look_J4/1
  Gain7/1 -> Mux80/2
  [q4] -> Mux80/1
  [q1] -> Mux81/1
  [qd1] -> Gain36/1
  Gain36/1 -> Mux81/2
  [q_dot] -> Mux82/1
  [qd1_dot] -> Mux82/2
  Mux82/1 -> rad2degree/1
  Mux81/1 -> Look_q1dot/1
  [e1] -> Look_q1dot/2
  rad2degree/1 -> Look_q1dot/3
  [q] -> q2qfdot_rad/2(q)
  q2qfdot_rad/2(qf_dot_next) -> Delay14/1, [q_dot]
  Delay14/1 -> q2qfdot_rad/4(qf_dot)
  q2qfdot_rad/1(qf_next) -> Delay15/1
  Delay15/1 -> q2qfdot_rad/3(qf)
  Constant49/1 -> Manual Switch25/2
  Constant73/1 -> Manual Switch25/1
  g_d2/1 -> Multiply/1
  Manual Switch25/1 -> Multiply1/2, Multiply/2
  g_d1/1 -> Multiply1/1
  run1/1 -> gripper/1
  break1/1 -> gripper/2
  gripper/1 -> HIL Write/5
  From140/1 -> To File22/1, Scope3/1
  From141/1 -> To File23/1, Scope3/2
  From143/1 -> To File14/1, Scope2/3
  From142/1 -> To File9/1, Scope2/2
  From144/1 -> To File8/1, Scope2/1
  Demux33/4 -> RBFNN_wrist/7(p2)
  Delay10/1 -> RBFNN_wrist/2(W_Q)
  Constant76/1 -> RBFNN_wrist/12(gamma_NN_Q)
  Constant81/1 -> RBFNN_wrist/11(gamma_NN_F)
  Constant78/1 -> RBFNN_wrist/14(eta_Q)
  RBFNN_wrist/4(W_Q_next) -> Delay10/1
  Demux31/4 -> RBFNN_wrist/5(z3)
  Demux32/4 -> RBFNN_wrist/6(p1)
  Demux30/4 -> RBFNN_wrist/4(z2)
  Constant77/1 -> RBFNN_wrist/13(eta_F)
  RBFNN_wrist/3(W_F_next) -> Scope19/1, Delay12/1
  RBFNN_wrist/1(U_F) -> Delay3/1
  Delay12/1 -> RBFNN_wrist/1(W_F)
  Manual Switch17/1 -> DIARC_new/2(switch_NN)
  Constant8/1 -> Manual Switch17/1
  Constant12/1 -> Manual Switch17/2
  [RBFNN] -> DIARC_new/3(RBFNN)
  [z2] -> Demux30/1
  [z3] -> Demux31/1
  [P_i] -> Demux32/1
  [P_o] -> Demux33/1
  RBFNN_wrist/6(look) -> Demux35/1
  DIARC_new/17(tolook_FLda1_joint3) -> Demux34/1
  Demux34/1 -> Scope17/1
  Demux34/2 -> Scope17/2
  Demux34/3 -> Scope17/3
  Demux34/4 -> Scope17/4
  From154/1 -> To File19/1, Scope18/1
  From153/1 -> Scope18/3, To File25/1
  From149/1 -> To File24/1, Scope18/2
  [qd4] -> RBFNN_wrist/8(qd)
  [qd4_dot] -> RBFNN_wrist/9(qd_dot)
  [qd4_dddot] -> RBFNN_wrist/10(qd_ddot)
  RBFNN_wrist/5(W_F_dot) -> Scope21/1
  Demux21/13 -> Mux47/4
  Demux21/14 -> Mux48/4
  Demux21/15 -> Mux49/4
  Demux21/16 -> Mux50/4
  [qd1_dot] -> Scope22/1
  [qd2_dot] -> Scope22/2
  [qd3_dot] -> Scope22/3
  [qd4_dot] -> Scope22/4
  [e4] -> RBFNN_wrist/3(z1)
  RBFNN_wrist/2(U_Q) -> Delay19/1
  Demux36/2 -> Scope25/2
  ? -> Mux84/4
  RBFNN_muti/2(U_Q) -> Delay20/1
  Mux84/1 -> Goto120/1
  RBFNN_muti/4(W_Q_next) -> Delay16/1
  From176/1 -> Mux89/1
  RBFNN_muti/3(W_F_next) -> Scope23/1, Delay17/1
  Delay20/1 -> Demux29/1
  Demux39/3 -> RBFNN_muti/6(p1)
  Constant74/1 -> RBFNN_muti/12(gamma_NN_Q)
  From175/1 -> Mux88/2
  From169/1 -> Demux39/1
  Delay18/1 -> Demux36/1
  Constant83/1 -> RBFNN_muti/11(gamma_NN_F)
  From166/1 -> Demux37/1
  Constant75/1 -> RBFNN_muti/13(eta_F)
  RBFNN_muti/6(look) -> Demux41/1
  RBFNN_muti/5(W_F_dot) -> Scope24/1
  RBFNN_muti/1(U_F) -> Delay18/1
  Demux37/3 -> RBFNN_muti/4(z2)
  Mux86/1 -> RBFNN_muti/3(z1)
  Demux38/3 -> RBFNN_muti/5(z3)
  Demux40/3 -> RBFNN_muti/7(p2)
  From168/1 -> Demux38/1
  Mux88/1 -> RBFNN_muti/8(qd)
  From177/1 -> Mux90/2
  Mux90/1 -> RBFNN_muti/10(qd_ddot)
  From171/1 -> Mux89/2
  Delay16/1 -> RBFNN_muti/2(W_Q)
  From172/1 -> Mux90/1
  From170/1 -> Demux40/1
  Delay17/1 -> RBFNN_muti/1(W_F)
  From173/1 -> Mux88/1
  ? -> Mux84/2
  Demux36/1 -> Mux84/1, Scope25/1
  Demux41/2 -> Scope26/2
  Demux29/2 -> Scope27/2
  Constant82/1 -> RBFNN_muti/14(eta_Q)
  Demux29/1 -> Mux84/3, Scope27/1
  Demux41/1 -> Scope26/1
  Mux89/1 -> RBFNN_muti/9(qd_dot)
  Demux43/3 -> RBFNN_smallarm/5(z3)
  Demux42/3 -> RBFNN_smallarm/4(z2)
  [qd3] -> RBFNN_smallarm/8(qd)
  [qd3_dot] -> RBFNN_smallarm/9(qd_dot)
  [qd3_dddot] -> RBFNN_smallarm/10(qd_ddot)
  Demux46/2 -> Scope31/2
  Demux46/1 -> Scope31/1
  Demux45/3 -> RBFNN_smallarm/7(p2)
  Constant86/1 -> RBFNN_smallarm/14(eta_Q)
  RBFNN_smallarm/5(W_F_dot) -> Scope29/1
  RBFNN_smallarm/6(look) -> Demux46/1
  Constant84/1 -> RBFNN_smallarm/12(gamma_NN_Q)
  Demux44/3 -> RBFNN_smallarm/6(p1)
  [P_o] -> Demux45/1
  [z2] -> Demux42/1
  RBFNN_smallarm/3(W_F_next) -> Scope28/1, Delay22/1
  [P_i] -> Demux44/1
  RBFNN_smallarm/1(U_F) -> Delay24/1
  Constant87/1 -> RBFNN_smallarm/11(gamma_NN_F)
  RBFNN_smallarm/2(U_Q) -> Delay23/1
  Delay22/1 -> RBFNN_smallarm/1(W_F)
  RBFNN_smallarm/4(W_Q_next) -> Delay21/1
  Delay21/1 -> RBFNN_smallarm/2(W_Q)
  Constant85/1 -> RBFNN_smallarm/13(eta_F)
  [z3] -> Demux43/1
  [e3] -> RBFNN_smallarm/3(z1)
  From167/1 -> Mux86/1
  From174/1 -> Mux86/2
  Mux83/1 -> [RBFNN_wrist]
  Mux85/1 -> [RBFNN_smallarm]
  [RBFNN_wrist] -> Mux87/1
  [RBFNN_smallarm] -> Mux87/2
  Mux87/1 -> [RBFNN]
  [P_i] -> Demux47/1
  [q3] -> To File40/1
  [q4] -> To File41/1
  [arc3] -> To File34/1
  [arc4] -> To File35/1
  Demux48/4 -> To File32/1
  [joint3_Qld] -> To File37/1
  Demux47/4 -> To File30/1
  [joint4_Qld] -> To File39/1
  Demux47/3 -> To File31/1
  [joint3_Fld] -> To File36/1
  [e4] -> To File27/1
  [P_o] -> Demux48/1
  [qd3] -> To File28/1
  [joint4_Fld] -> To File38/1
  [e3] -> To File26/1
  Demux48/3 -> To File33/1
  [qd4] -> To File29/1
  [qd4_dot] -> To File43/1
  [qd3_dot] -> To File42/1
  From214/1 -> To File61/1
  From213/1 -> To File60/1
  Demux50/3 -> To File51/1
  From210/1 -> To File47/1
  From206/1 -> To File57/1
  From212/1 -> Demux50/1
  From203/1 -> To File54/1
  From209/1 -> To File46/1
  From199/1 -> To File44/1
  Demux49/3 -> To File49/1
  From204/1 -> To File56/1
  Demux50/4 -> To File50/1
  From207/1 -> To File58/1
  From201/1 -> To File52/1
  Demux49/4 -> To File48/1
  From211/1 -> Demux49/1
  From205/1 -> To File55/1
  From200/1 -> To File45/1
  From208/1 -> To File59/1
  From202/1 -> To File53/1
  Delay19/1 -> Mux83/2, Scope5/2, To File67/1
  Delay3/1 -> To File66/1, Mux83/1, Scope5/1
  Delay24/1 -> Mux85/1, To File62/1, Scope30/1
  Delay23/1 -> Mux85/2, To File63/1, Scope30/2
  Demux51/1 -> Scope32/1
  Demux51/2 -> Scope32/2
  Demux51/3 -> Scope32/3
  Demux51/4 -> Scope32/4
  Demux51/5 -> Scope32/5
  Demux35/1 -> Scope6/1
  Demux35/2 -> Scope6/2
  Demux35/3 -> Scope6/3
  Demux35/4 -> Scope6/4
  Demux35/5 -> Scope6/5
  Demux52/3 -> Scope33/3
  Demux52/2 -> Scope33/2
  Demux52/5 -> Scope33/5
  Demux52/1 -> Scope33/1
  Demux52/4 -> Scope33/4
